simulink model "CORDIC"  (R2021a)
settings: Solver=VariableStepAuto  StartTime=0.0  StopTime=400  RelTol=1e-3
undefined symbols (not defined in the file or in its folder): AXI4, Lite
libraries: hdlBasic x776, xbsIndex_r4 x1
(part 1 of 7)
settings Model: Creator=jz118  LastModifiedBy=jz118

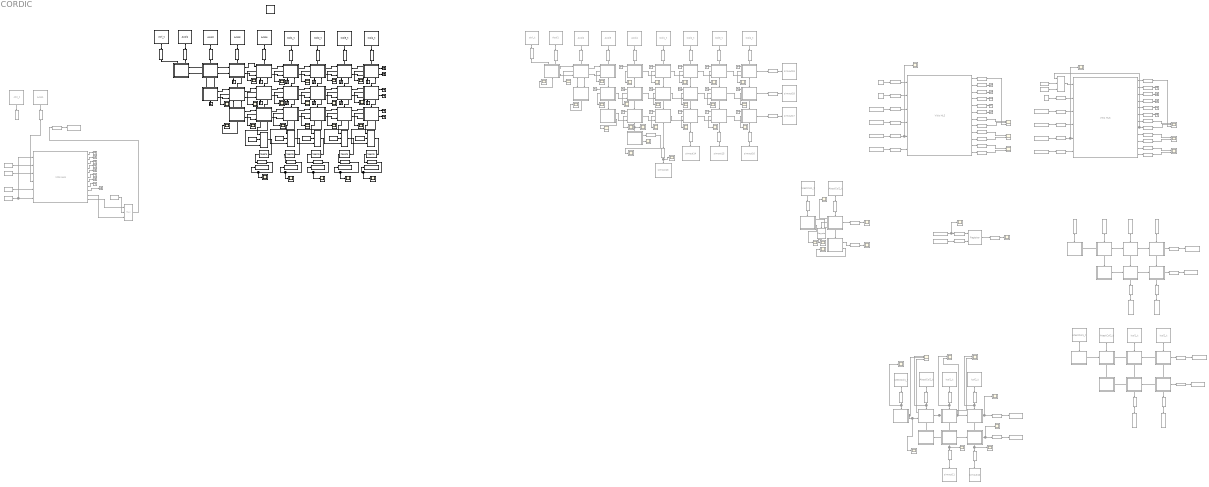
== system CORDIC ==
  " System Generator1" : xbsIndex_r4/ System Generator  Tag=genX  xilinxfamily=zynq  part=xc7z020  speed=-1  package=clg484  synthesis_tool=Vivado  clock_wrapper=Clock Enables  directory=./netlistA4  proj_type=Vivado  Synth_file=Vivado Synthesis Defaults  Impl_file=Vivado Implementation Defaults  testbench=off  simulink_period=1  sysclk_period=10  dcm_input_clock_period=10  incr_netlist=off  trim_vbits=Everywhere in SubSystem  dbl_ovrd=According to Block Masks  core_generation=According to Block Masks  run_coregen=off  deprecated_control=off  eval_field=0  block_type=sysgen
  Constant : hdlBasic/Constant  Commented=on  const=0  gui_display_data_type=Boolean  arith_type=Boolean  n_bits=16  bin_pt=14  preci_type=Single  exp_width=8  frac_width=24  explicit_period=off  period=1  XmcBlockStatus=1  maskContainerNames=tabcontainer1  block_type=constant  block_config=sysgen:Constant_config
  Constant1 : hdlBasic/Constant  Commented=on  const=1.0  gui_display_data_type=Boolean  arith_type=Boolean  n_bits=16  bin_pt=14  preci_type=Single  exp_width=8  frac_width=24  explicit_period=off  period=1  XmcBlockStatus=1  maskContainerNames=tabcontainer1  block_type=constant  block_config=sysgen:Constant_config
  Constant10 : hdlBasic/Constant  Commented=on  const=0  gui_display_data_type=Fixed-point  arith_type=Signed (2's comp)  n_bits=16  bin_pt=13  preci_type=Single  exp_width=8  frac_width=24  explicit_period=off  period=1  XmcBlockStatus=1  maskContainerNames=tabcontainer1  block_type=constant  block_config=sysgen:Constant_config
  Constant{4,6..8,11} (5 alike) : hdlBasic/Constant  const=0  gui_display_data_type=Fixed-point  arith_type=Signed (2's comp)  n_bits=16  bin_pt=13  preci_type=Single  exp_width=8  frac_width=24  explicit_period=off  period=1  XmcBlockStatus=1  maskContainerNames=tabcontainer1  block_type=constant  block_config=sysgen:Constant_config
  Constant12 : hdlBasic/Constant  Commented=on  const=0  gui_display_data_type=Boolean  arith_type=Boolean  n_bits=16  bin_pt=13  preci_type=Single  exp_width=8  frac_width=24  explicit_period=off  period=1  XmcBlockStatus=1  maskContainerNames=tabcontainer1  block_type=constant  block_config=sysgen:Constant_config
  Constant13 : hdlBasic/Constant  Commented=on  const=1  gui_display_data_type=Boolean  arith_type=Boolean  n_bits=16  bin_pt=13  preci_type=Single  exp_width=8  frac_width=24  explicit_period=off  period=1  XmcBlockStatus=1  maskContainerNames=tabcontainer1  block_type=constant  block_config=sysgen:Constant_config
  Constant14 : hdlBasic/Constant  Commented=on  const=0  gui_display_data_type=Fixed-point  arith_type=Signed (2's comp)  n_bits=16  bin_pt=13  preci_type=Single  exp_width=8  frac_width=24  explicit_period=off  period=1  XmcBlockStatus=1  maskContainerNames=tabcontainer1  block_type=constant  block_config=sysgen:Constant_config
  Constant2 : Constant  Commented=on
  Constant3 : Constant  Commented=on  Value=0
  Constant5 : Constant  Commented=on
  Constant9 : hdlBasic/Constant  Commented=on  const=0  gui_display_data_type=Fixed-point  arith_type=Signed (2's comp)  n_bits=16  bin_pt=13  preci_type=Single  exp_width=8  frac_width=24  explicit_period=off  period=1  XmcBlockStatus=1  maskContainerNames=tabcontainer1  block_type=constant  block_config=sysgen:Constant_config
  From Workspace1 : FromWorkspace  Commented=on  VariableName=y
  From Workspace10 : FromWorkspace  Commented=on  VariableName=AtestCol2_t
  From Workspace11 : FromWorkspace  Commented=on  VariableName=y
  From Workspace12 : FromWorkspace  Commented=on  VariableName=mode
  From Workspace13 : FromWorkspace  Commented=on  VariableName=theta
  From Workspace14 : FromWorkspace  Commented=on  VariableName=x
  From Workspace15 : FromWorkspace  Commented=on  VariableName=Icol1_t
  From Workspace16 : FromWorkspace  Commented=on  VariableName=Icol2_t
  From Workspace17 : FromWorkspace  Commented=on  VariableName=AtestCol1_t
  From Workspace18 : FromWorkspace  Commented=on  VariableName=AtestCol2_t
  From Workspace19 : FromWorkspace  Commented=on  VariableName=Icol1_t
  From Workspace2 : FromWorkspace  Commented=on  VariableName=mode
  From Workspace20 : FromWorkspace  Commented=on  VariableName=Icol2_t
  From Workspace21 : FromWorkspace  Commented=on  VariableName=regenable
  From Workspace22 : FromWorkspace  Commented=on  VariableName=regtest
  From Workspace23 : FromWorkspace  Commented=on  VariableName=AtestCol1_t
  From Workspace24 : FromWorkspace  Commented=on  VariableName=AtestCol2_t
  From Workspace25 : FromWorkspace  Commented=on  VariableName=Acol1
  From Workspace26 : FromWorkspace  Commented=on  VariableName=Acol2
  From Workspace27 : FromWorkspace  Commented=on  VariableName=Acol3
  From Workspace28 : FromWorkspace  Commented=on  VariableName=Acol4
  From Workspace29 : FromWorkspace  Commented=on  VariableName=Icol1_t
  From Workspace3 : FromWorkspace  Commented=on  VariableName=theta
  From Workspace30 : FromWorkspace  Commented=on  VariableName=Icol2_t
  From Workspace31 : FromWorkspace  Commented=on  VariableName=Icol3_t
  From Workspace32 : FromWorkspace  Commented=on  VariableName=Icol4_t
  From Workspace33 : FromWorkspace  Commented=on  VariableName=ctrl_t
  From Workspace34 : FromWorkspace  VariableName=Acol1
  From Workspace35 : FromWorkspace  VariableName=Acol2
  From Workspace36 : FromWorkspace  VariableName=Acol3
  From Workspace37 : FromWorkspace  VariableName=Acol4
  From Workspace38 : FromWorkspace  VariableName=ctrl_t
  From Workspace39 : FromWorkspace  VariableName=Icol1_t
  From Workspace4 : FromWorkspace  Commented=on  VariableName=x
  From Workspace40 : FromWorkspace  VariableName=Icol2_t
  From Workspace41 : FromWorkspace  VariableName=Icol3_t
  From Workspace42 : FromWorkspace  VariableName=Icol4_t
  From Workspace43 : FromWorkspace  Commented=on  VariableName=Acol1
  From Workspace44 : FromWorkspace  Commented=on  VariableName=ctrl_t
  From Workspace5 : FromWorkspace  Commented=on  VariableName=col1
  From Workspace6 : FromWorkspace  Commented=on  VariableName=col2
  From Workspace7 : FromWorkspace  Commented=on  VariableName=ident1
  From Workspace8 : FromWorkspace  Commented=on  VariableName=ident2
  From Workspace9 : FromWorkspace  Commented=on  VariableName=AtestCol1_t
  Gateway In{1,5,9..11} (5 alike) : hdlBasic/Gateway In  Commented=on  gui_display_data_type=Boolean  arith_type=Boolean  n_bits=16  bin_pt=3  preci_type=Single  exp_width=8  frac_width=24  rows=1  columns=1  quantization="Round  (unbiased: +/- Inf)"  overflow=Saturate  period=1  UseAsADC=off  ADCChannel='1'  interface=None  automatic_assignment=on  address_offset=hex2dec('00')  intf_name=''  intf_description=''  default_value=0  timing_constraint=None  locs_specified=off  LOCs={}  io_standard={}  inherit_from_input=off  hdl_port=on  XmcBlockStatus=1  maskContainerNames=group4  block_type=gatewayin  block_config=sysgen:gateway_in_config  block_width_w=590  block_height_w=620  block_width=640  block_height=850
  Gateway In{2..4,6..8,12..15,17..27} (21 alike) : hdlBasic/Gateway In  Commented=on  gui_display_data_type=Fixed-point  arith_type=Signed (2's comp)  n_bits=16  bin_pt=13  preci_type=Single  exp_width=8  frac_width=24  rows=1  columns=1  quantization="Round  (unbiased: +/- Inf)"  overflow=Saturate  period=1  UseAsADC=off  ADCChannel='1'  interface=None  automatic_assignment=on  address_offset=hex2dec('00')  intf_name=''  intf_description=''  default_value=0  timing_constraint=None  locs_specified=off  LOCs={}  io_standard={}  inherit_from_input=off  hdl_port=on  XmcBlockStatus=1  maskContainerNames=group4  block_type=gatewayin  block_config=sysgen:gateway_in_config  block_width_w=590  block_height_w=620  block_width=640  block_height=850
  Gateway In16 : hdlBasic/Gateway In  Commented=on  gui_display_data_type=Boolean  arith_type=Boolean  n_bits=16  bin_pt=13  preci_type=Single  exp_width=8  frac_width=24  rows=1  columns=1  quantization="Round  (unbiased: +/- Inf)"  overflow=Saturate  period=1  UseAsADC=off  ADCChannel='1'  interface=None  automatic_assignment=on  address_offset=hex2dec('00')  intf_name=''  intf_description=''  default_value=0  timing_constraint=None  locs_specified=off  LOCs={}  io_standard={}  inherit_from_input=off  hdl_port=on  XmcBlockStatus=1  maskContainerNames=group4  block_type=gatewayin  block_config=sysgen:gateway_in_config  block_width_w=590  block_height_w=620  block_width=640  block_height=850
  Gateway In28 : hdlBasic/Gateway In  Commented=on  gui_display_data_type=Boolean  arith_type=Boolean  n_bits=16  bin_pt=13  preci_type=Single  exp_width=8  frac_width=24  rows=1  columns=1  quantization="Round  (unbiased: +/- Inf)"  overflow=Saturate  period=1  UseAsADC=off  ADCChannel='1'  interface=None  automatic_assignment=on  address_offset=hex2dec('00')  intf_name=''  intf_description=''  default_value=0  timing_constraint=None  locs_specified=off  LOCs={}  io_standard={}  inherit_from_input=off  hdl_port=on  XmcBlockStatus=1  maskContainerNames=group4  block_type=gatewayin  block_config=sysgen:gateway_in_config  block_width_w=590  block_height_w=620  block_width=640  block_height=850
  Gateway In29 : hdlBasic/Gateway In  gui_display_data_type=Fixed-point  arith_type=Signed (2's comp)  n_bits=16  bin_pt=13  preci_type=Single  exp_width=8  frac_width=24  rows=1  columns=1  quantization="Round  (unbiased: +/- Inf)"  overflow=Saturate  period=1  UseAsADC=off  ADCChannel='1'  interface=AXI4-Lite  automatic_assignment=on  address_offset=hex2dec('00')  intf_name=''  intf_description='Acol1'  default_value=0  timing_constraint=None  locs_specified=off  LOCs={}  io_standard={}  inherit_from_input=off  hdl_port=on  XmcBlockStatus=1  maskContainerNames=group4  block_type=gatewayin  block_config=sysgen:gateway_in_config  block_width_w=590  block_height_w=620  block_width=640  block_height=850
  Gateway In30 : hdlBasic/Gateway In  gui_display_data_type=Fixed-point  arith_type=Signed (2's comp)  n_bits=16  bin_pt=13  preci_type=Single  exp_width=8  frac_width=24  rows=1  columns=1  quantization="Round  (unbiased: +/- Inf)"  overflow=Saturate  period=1  UseAsADC=off  ADCChannel='1'  interface=AXI4-Lite  automatic_assignment=on  address_offset=hex2dec('00')  intf_name=''  intf_description='Acol2'  default_value=0  timing_constraint=None  locs_specified=off  LOCs={}  io_standard={}  inherit_from_input=off  hdl_port=on  XmcBlockStatus=1  maskContainerNames=group4  block_type=gatewayin  block_config=sysgen:gateway_in_config  block_width_w=590  block_height_w=620  block_width=640  block_height=850
  Gateway In31 : hdlBasic/Gateway In  gui_display_data_type=Fixed-point  arith_type=Signed (2's comp)  n_bits=16  bin_pt=13  preci_type=Single  exp_width=8  frac_width=24  rows=1  columns=1  quantization="Round  (unbiased: +/- Inf)"  overflow=Saturate  period=1  UseAsADC=off  ADCChannel='1'  interface=AXI4-Lite  automatic_assignment=on  address_offset=hex2dec('00')  intf_name=''  intf_description='Acol3'  default_value=0  timing_constraint=None  locs_specified=off  LOCs={}  io_standard={}  inherit_from_input=off  hdl_port=on  XmcBlockStatus=1  maskContainerNames=group4  block_type=gatewayin  block_config=sysgen:gateway_in_config  block_width_w=590  block_height_w=620  block_width=640  block_height=850
  Gateway In32 : hdlBasic/Gateway In  gui_display_data_type=Fixed-point  arith_type=Signed (2's comp)  n_bits=16  bin_pt=13  preci_type=Single  exp_width=8  frac_width=24  rows=1  columns=1  quantization="Round  (unbiased: +/- Inf)"  overflow=Saturate  period=1  UseAsADC=off  ADCChannel='1'  interface=AXI4-Lite  automatic_assignment=on  address_offset=hex2dec('00')  intf_name=''  intf_description='Acol4'  default_value=0  timing_constraint=None  locs_specified=off  LOCs={}  io_standard={}  inherit_from_input=off  hdl_port=on  XmcBlockStatus=1  maskContainerNames=group4  block_type=gatewayin  block_config=sysgen:gateway_in_config  block_width_w=590  block_height_w=620  block_width=640  block_height=850
  Gateway In33 : hdlBasic/Gateway In  Commented=on  gui_display_data_type=Fixed-point  arith_type=Signed (2's comp)  n_bits=16  bin_pt=13  preci_type=Single  exp_width=8  frac_width=24  rows=1  columns=1  quantization="Round  (unbiased: +/- Inf)"  overflow=Saturate  period=1  UseAsADC=off  ADCChannel='1'  interface=AXI4-Lite  automatic_assignment=on  address_offset=hex2dec('00')  intf_name=''  intf_description='Acol1'  default_value=0  timing_constraint=None  locs_specified=off  LOCs={}  io_standard={}  inherit_from_input=off  hdl_port=on  XmcBlockStatus=1  maskContainerNames=group4  block_type=gatewayin  block_config=sysgen:gateway_in_config  block_width_w=590  block_height_w=620  block_width=640  block_height=850
  Gateway In34 : hdlBasic/Gateway In  gui_display_data_type=Fixed-point  arith_type=Signed (2's comp)  n_bits=16  bin_pt=13  preci_type=Single  exp_width=8  frac_width=24  rows=1  columns=1  quantization="Round  (unbiased: +/- Inf)"  overflow=Saturate  period=1  UseAsADC=off  ADCChannel='1'  interface=AXI4-Lite  automatic_assignment=on  address_offset=hex2dec('00')  intf_name=''  intf_description='Icol1_t'  default_value=0  timing_constraint=None  locs_specified=off  LOCs={}  io_standard={}  inherit_from_input=off  hdl_port=on  XmcBlockStatus=1  maskContainerNames=group4  block_type=gatewayin  block_config=sysgen:gateway_in_config  block_width_w=590  block_height_w=620  block_width=640  block_height=850
  Gateway In35 : hdlBasic/Gateway In  gui_display_data_type=Fixed-point  arith_type=Signed (2's comp)  n_bits=16  bin_pt=13  preci_type=Single  exp_width=8  frac_width=24  rows=1  columns=1  quantization="Round  (unbiased: +/- Inf)"  overflow=Saturate  period=1  UseAsADC=off  ADCChannel='1'  interface=AXI4-Lite  automatic_assignment=on  address_offset=hex2dec('00')  intf_name=''  intf_description='Icol2_t'  default_value=0  timing_constraint=None  locs_specified=off  LOCs={}  io_standard={}  inherit_from_input=off  hdl_port=on  XmcBlockStatus=1  maskContainerNames=group4  block_type=gatewayin  block_config=sysgen:gateway_in_config  block_width_w=590  block_height_w=620  block_width=640  block_height=850
  Gateway In36 : hdlBasic/Gateway In  gui_display_data_type=Fixed-point  arith_type=Signed (2's comp)  n_bits=16  bin_pt=13  preci_type=Single  exp_width=8  frac_width=24  rows=1  columns=1  quantization="Round  (unbiased: +/- Inf)"  overflow=Saturate  period=1  UseAsADC=off  ADCChannel='1'  interface=AXI4-Lite  automatic_assignment=on  address_offset=hex2dec('00')  intf_name=''  intf_description='Icol3_t'  default_value=0  timing_constraint=None  locs_specified=off  LOCs={}  io_standard={}  inherit_from_input=off  hdl_port=on  XmcBlockStatus=1  maskContainerNames=group4  block_type=gatewayin  block_config=sysgen:gateway_in_config  block_width_w=590  block_height_w=620  block_width=640  block_height=850
  Gateway In37 : hdlBasic/Gateway In  gui_display_data_type=Fixed-point  arith_type=Signed (2's comp)  n_bits=16  bin_pt=13  preci_type=Single  exp_width=8  frac_width=24  rows=1  columns=1  quantization="Round  (unbiased: +/- Inf)"  overflow=Saturate  period=1  UseAsADC=off  ADCChannel='1'  interface=AXI4-Lite  automatic_assignment=on  address_offset=hex2dec('00')  intf_name=''  intf_description='Icol4_t'  default_value=0  timing_constraint=None  locs_specified=off  LOCs={}  io_standard={}  inherit_from_input=off  hdl_port=on  XmcBlockStatus=1  maskContainerNames=group4  block_type=gatewayin  block_config=sysgen:gateway_in_config  block_width_w=590  block_height_w=620  block_width=640  block_height=850
  Gateway Out{,1..42,44..47} (47 alike) : hdlBasic/Gateway Out  Commented=on  inherit_from_input=off  hdl_port=on  rows=1  columns=1  UseAsDAC=off  DACChannel='1'  interface=None  automatic_assignment=on  address_offset=hex2dec('00')  intf_name=''  intf_description=''  timing_constraint=None  locs_specified=off  LOCs={}  io_standard={}  XmcBlockStatus=1  maskContainerNames=group4  block_type=gatewayout  block_config=sysgen:gateway_out_config  block_width_w=590  block_height_w=620  block_width=620  block_height=750
  Gateway Out43 : hdlBasic/Gateway Out  inherit_from_input=off  hdl_port=on  rows=1  columns=1  UseAsDAC=off  DACChannel='1'  interface=AXI4-Lite  automatic_assignment=on  address_offset=hex2dec('00')  intf_name=''  intf_description='R_4_4'  timing_constraint=None  locs_specified=off  LOCs={}  io_standard={}  XmcBlockStatus=1  maskContainerNames=group4  block_type=gatewayout  block_config=sysgen:gateway_out_config  block_width_w=590  block_height_w=620  block_width=620  block_height=750
  Gateway Out48 : hdlBasic/Gateway Out  inherit_from_input=off  hdl_port=on  rows=1  columns=1  UseAsDAC=off  DACChannel='1'  interface=AXI4-Lite  automatic_assignment=on  address_offset=hex2dec('00')  intf_name=''  intf_description='Q_4_1'  timing_constraint=None  locs_specified=off  LOCs={}  io_standard={}  XmcBlockStatus=1  maskContainerNames=group4  block_type=gatewayout  block_config=sysgen:gateway_out_config  block_width_w=590  block_height_w=620  block_width=620  block_height=750
  Gateway Out49 : hdlBasic/Gateway Out  inherit_from_input=off  hdl_port=on  rows=1  columns=1  UseAsDAC=off  DACChannel='1'  interface=AXI4-Lite  automatic_assignment=on  address_offset=hex2dec('00')  intf_name=''  intf_description='Q_4_2'  timing_constraint=None  locs_specified=off  LOCs={}  io_standard={}  XmcBlockStatus=1  maskContainerNames=group4  block_type=gatewayout  block_config=sysgen:gateway_out_config  block_width_w=590  block_height_w=620  block_width=620  block_height=750
  Gateway Out50 : hdlBasic/Gateway Out  inherit_from_input=off  hdl_port=on  rows=1  columns=1  UseAsDAC=off  DACChannel='1'  interface=AXI4-Lite  automatic_assignment=on  address_offset=hex2dec('00')  intf_name=''  intf_description='Q_4_3'  timing_constraint=None  locs_specified=off  LOCs={}  io_standard={}  XmcBlockStatus=1  maskContainerNames=group4  block_type=gatewayout  block_config=sysgen:gateway_out_config  block_width_w=590  block_height_w=620  block_width=620  block_height=750
  Gateway Out51 : hdlBasic/Gateway Out  inherit_from_input=off  hdl_port=on  rows=1  columns=1  UseAsDAC=off  DACChannel='1'  interface=AXI4-Lite  automatic_assignment=on  address_offset=hex2dec('00')  intf_name=''  intf_description='Q_4_4'  timing_constraint=None  locs_specified=off  LOCs={}  io_standard={}  XmcBlockStatus=1  maskContainerNames=group4  block_type=gatewayout  block_config=sysgen:gateway_out_config  block_width_w=590  block_height_w=620  block_width=620  block_height=750
  Gateway Out52 : hdlBasic/Gateway Out  Commented=on  inherit_from_input=off  hdl_port=on  rows=1  columns=1  UseAsDAC=off  DACChannel='1'  interface=AXI4-Lite  automatic_assignment=on  address_offset=hex2dec('00')  intf_name=''  intf_description='R_4_4'  timing_constraint=None  locs_specified=off  LOCs={}  io_standard={}  XmcBlockStatus=1  maskContainerNames=group4  block_type=gatewayout  block_config=sysgen:gateway_out_config  block_width_w=590  block_height_w=620  block_width=620  block_height=750
  Mux : hdlBasic/Mux  Commented=on  inputs=2  en=off  latency=1  precision=Full  arith_type=Unsigned  n_bits=16  bin_pt=14  quantization=Truncate  overflow=Wrap  XmcBlockStatus=1  maskContainerNames=tabcontainer1  block_type=mux  block_config=sysgen:Mux_config
  Mux{1..5} (5 alike) : hdlBasic/Mux  inputs=2  en=off  latency=1  precision=Full  arith_type=Unsigned  n_bits=16  bin_pt=14  quantization=Truncate  overflow=Wrap  XmcBlockStatus=1  maskContainerNames=tabcontainer1  block_type=mux  block_config=sysgen:Mux_config
  Mux6 : hdlBasic/Mux  Commented=on  inputs=2  en=off  latency=1  precision=Full  arith_type=Unsigned  n_bits=16  bin_pt=14  quantization=Truncate  overflow=Wrap  XmcBlockStatus=1  maskContainerNames=tabcontainer1  block_type=mux  block_config=sysgen:Mux_config
  Negate : hdlBasic/Negate  Commented=on  precision=Full  arith_type=Unsigned  n_bits=16  bin_pt=14  quantization=Truncate  overflow=Wrap  en=off  latency=0  XmcBlockStatus=1  maskContainerNames=tabcontainer1  block_type=negate  block_config=sysgen:Negate_config
  Negate{1..5} (5 alike) : hdlBasic/Negate  precision=Full  arith_type=Unsigned  n_bits=16  bin_pt=14  quantization=Truncate  overflow=Wrap  en=off  latency=0  XmcBlockStatus=1  maskContainerNames=tabcontainer1  block_type=negate  block_config=sysgen:Negate_config
  Register : hdlBasic/Register  Commented=on  init=0  rst=off  en=on  XmcBlockStatus=1  maskContainerNames=tabcontainer1  block_type=register  block_config=sysgen:Register_config
  Rotation : Subsystem  Commented=on
      settings: PortSchema="{\"entries\":[{\"content\":{\"sides\":[{\"content\":{\"connectorIds\":[\"In1\"]},\"type\":\"ConnectorPlacement.EquallySpacedRectSide\",\"uuid\":\"b989bfd3-647b-468d-a24b-67c5817c2fb9\"},{\"content\":{\"connectorIds\":[\"Out1\"],\"side\":\"RIGHT\"},\"type\":\"ConnectorPlacement.EquallySpacedRectSide\",\"uuid\":\"15839450-c6b9-4b4c-b490-793a0225ad70\"},{\"content\":{\"connectorIds\":[\"In2\"],\"side\":\"TOP\"},\"type\":\"ConnectorPlacement.EquallySpacedRectSide\",\"uuid\":\"69a0ff69-1754-49ce-bc12-3d58954b90b5\"},{\"content\":{\"connectorIds\":[\"Out2\"],\"side\":\"BOTTOM\"},\"type\":\"ConnectorPlacement.EquallySpacedRectSide\",\"uuid\":\"c7c95c77-bae3-47b7-a54f-9afc9f4e7b60\"}]},\"type\":\"ConnectorPlacement.EquallySpacedConnector\",\"uuid\":\"47487c21-2009-4dc3-9515-f1b42d882620\"}],\"packageUris\":[\"http://schema.mathworks.com/mf0/Connector/R2020b\"],\"version\":\"1.0\"}"
  Rotation1 : Subsystem  Commented=on
      settings: PortSchema="{\"entries\":[{\"content\":{\"sides\":[{\"content\":{\"connectorIds\":[\"In1\"]},\"type\":\"ConnectorPlacement.EquallySpacedRectSide\",\"uuid\":\"b989bfd3-647b-468d-a24b-67c5817c2fb9\"},{\"content\":{\"connectorIds\":[\"Out1\"],\"side\":\"RIGHT\"},\"type\":\"ConnectorPlacement.EquallySpacedRectSide\",\"uuid\":\"15839450-c6b9-4b4c-b490-793a0225ad70\"},{\"content\":{\"connectorIds\":[\"In2\"],\"side\":\"TOP\"},\"type\":\"ConnectorPlacement.EquallySpacedRectSide\",\"uuid\":\"69a0ff69-1754-49ce-bc12-3d58954b90b5\"},{\"content\":{\"connectorIds\":[\"Out2\"],\"side\":\"BOTTOM\"},\"type\":\"ConnectorPlacement.EquallySpacedRectSide\",\"uuid\":\"c7c95c77-bae3-47b7-a54f-9afc9f4e7b60\"}]},\"type\":\"ConnectorPlacement.EquallySpacedConnector\",\"uuid\":\"47487c21-2009-4dc3-9515-f1b42d882620\"}],\"packageUris\":[\"http://schema.mathworks.com/mf0/Connector/R2020b\"],\"version\":\"1.0\"}"
  Rotation10 : Subsystem  Commented=on
      settings: PortSchema="{\"entries\":[{\"content\":{\"sides\":[{\"content\":{\"connectorIds\":[\"Out3\",\"In1\"]},\"type\":\"ConnectorPlacement.EquallySpacedRectSide\",\"uuid\":\"b989bfd3-647b-468d-a24b-67c5817c2fb9\"},{\"content\":{\"connectorIds\":[\"Out1\"],\"side\":\"RIGHT\"},\"type\":\"ConnectorPlacement.EquallySpacedRectSide\",\"uuid\":\"15839450-c6b9-4b4c-b490-793a0225ad70\"},{\"content\":{\"connectorIds\":[\"In2\"],\"side\":\"TOP\"},\"type\":\"ConnectorPlacement.EquallySpacedRectSide\",\"uuid\":\"69a0ff69-1754-49ce-bc12-3d58954b90b5\"},{\"content\":{\"connectorIds\":[\"Out2\"],\"side\":\"BOTTOM\"},\"type\":\"ConnectorPlacement.EquallySpacedRectSide\",\"uuid\":\"c7c95c77-bae3-47b7-a54f-9afc9f4e7b60\"}]},\"type\":\"ConnectorPlacement.EquallySpacedConnector\",\"uuid\":\"47487c21-2009-4dc3-9515-f1b42d882620\"}],\"packageUris\":[\"http://schema.mathworks.com/mf0/Connector/R2020b\"],\"version\":\"1.0\"}"
  Rotation11 : Subsystem  Commented=on
      settings: PortSchema="{\"entries\":[{\"content\":{\"sides\":[{\"content\":{\"connectorIds\":[\"In1\"]},\"type\":\"ConnectorPlacement.EquallySpacedRectSide\",\"uuid\":\"b989bfd3-647b-468d-a24b-67c5817c2fb9\"},{\"content\":{\"connectorIds\":[\"Out1\"],\"side\":\"RIGHT\"},\"type\":\"ConnectorPlacement.EquallySpacedRectSide\",\"uuid\":\"15839450-c6b9-4b4c-b490-793a0225ad70\"},{\"content\":{\"connectorIds\":[\"In2\"],\"side\":\"TOP\"},\"type\":\"ConnectorPlacement.EquallySpacedRectSide\",\"uuid\":\"69a0ff69-1754-49ce-bc12-3d58954b90b5\"},{\"content\":{\"connectorIds\":[\"Out2\"],\"side\":\"BOTTOM\"},\"type\":\"ConnectorPlacement.EquallySpacedRectSide\",\"uuid\":\"c7c95c77-bae3-47b7-a54f-9afc9f4e7b60\"}]},\"type\":\"ConnectorPlacement.EquallySpacedConnector\",\"uuid\":\"47487c21-2009-4dc3-9515-f1b42d882620\"}],\"packageUris\":[\"http://schema.mathworks.com/mf0/Connector/R2020b\"],\"version\":\"1.0\"}"
  Rotation12 : Subsystem  Commented=on
      settings: PortSchema="{\"entries\":[{\"content\":{\"sides\":[{\"content\":{\"connectorIds\":[\"In1\"]},\"type\":\"ConnectorPlacement.EquallySpacedRectSide\",\"uuid\":\"b989bfd3-647b-468d-a24b-67c5817c2fb9\"},{\"content\":{\"connectorIds\":[\"Out1\"],\"side\":\"RIGHT\"},\"type\":\"ConnectorPlacement.EquallySpacedRectSide\",\"uuid\":\"15839450-c6b9-4b4c-b490-793a0225ad70\"},{\"content\":{\"connectorIds\":[\"In2\"],\"side\":\"TOP\"},\"type\":\"ConnectorPlacement.EquallySpacedRectSide\",\"uuid\":\"69a0ff69-1754-49ce-bc12-3d58954b90b5\"},{\"content\":{\"connectorIds\":[\"Out2\"],\"side\":\"BOTTOM\"},\"type\":\"ConnectorPlacement.EquallySpacedRectSide\",\"uuid\":\"c7c95c77-bae3-47b7-a54f-9afc9f4e7b60\"}]},\"type\":\"ConnectorPlacement.EquallySpacedConnector\",\"uuid\":\"47487c21-2009-4dc3-9515-f1b42d882620\"}],\"packageUris\":[\"http://schema.mathworks.com/mf0/Connector/R2020b\"],\"version\":\"1.0\"}"
  Rotation13 : Subsystem  Commented=on
      settings: PortSchema="{\"entries\":[{\"content\":{\"sides\":[{\"content\":{\"connectorIds\":[\"Out3\",\"Out4\",\"In1\"]},\"type\":\"ConnectorPlacement.EquallySpacedRectSide\",\"uuid\":\"b989bfd3-647b-468d-a24b-67c5817c2fb9\"},{\"content\":{\"connectorIds\":[\"Out1\"],\"side\":\"RIGHT\"},\"type\":\"ConnectorPlacement.EquallySpacedRectSide\",\"uuid\":\"15839450-c6b9-4b4c-b490-793a0225ad70\"},{\"content\":{\"connectorIds\":[\"In2\"],\"side\":\"TOP\"},\"type\":\"ConnectorPlacement.EquallySpacedRectSide\",\"uuid\":\"69a0ff69-1754-49ce-bc12-3d58954b90b5\"},{\"content\":{\"connectorIds\":[\"Out2\"],\"side\":\"BOTTOM\"},\"type\":\"ConnectorPlacement.EquallySpacedRectSide\",\"uuid\":\"c7c95c77-bae3-47b7-a54f-9afc9f4e7b60\"}]},\"type\":\"ConnectorPlacement.EquallySpacedConnector\",\"uuid\":\"47487c21-2009-4dc3-9515-f1b42d882620\"}],\"packageUris\":[\"http://schema.mathworks.com/mf0/Connector/R2020b\"],\"version\":\"1.0\"}"
  Rotation14 : Subsystem  Commented=on
      settings: PortSchema="{\"entries\":[{\"content\":{\"sides\":[{\"content\":{\"connectorIds\":[\"In1\"]},\"type\":\"ConnectorPlacement.EquallySpacedRectSide\",\"uuid\":\"b989bfd3-647b-468d-a24b-67c5817c2fb9\"},{\"content\":{\"connectorIds\":[\"Out1\"],\"side\":\"RIGHT\"},\"type\":\"ConnectorPlacement.EquallySpacedRectSide\",\"uuid\":\"15839450-c6b9-4b4c-b490-793a0225ad70\"},{\"content\":{\"connectorIds\":[\"In2\"],\"side\":\"TOP\"},\"type\":\"ConnectorPlacement.EquallySpacedRectSide\",\"uuid\":\"69a0ff69-1754-49ce-bc12-3d58954b90b5\"},{\"content\":{\"connectorIds\":[\"Out2\"],\"side\":\"BOTTOM\"},\"type\":\"ConnectorPlacement.EquallySpacedRectSide\",\"uuid\":\"c7c95c77-bae3-47b7-a54f-9afc9f4e7b60\"}]},\"type\":\"ConnectorPlacement.EquallySpacedConnector\",\"uuid\":\"47487c21-2009-4dc3-9515-f1b42d882620\"}],\"packageUris\":[\"http://schema.mathworks.com/mf0/Connector/R2020b\"],\"version\":\"1.0\"}"
  Rotation15 : Subsystem  Commented=on
      settings: PortSchema="{\"entries\":[{\"content\":{\"sides\":[{\"content\":{\"connectorIds\":[\"In1\"]},\"type\":\"ConnectorPlacement.EquallySpacedRectSide\",\"uuid\":\"b989bfd3-647b-468d-a24b-67c5817c2fb9\"},{\"content\":{\"connectorIds\":[\"Out1\"],\"side\":\"RIGHT\"},\"type\":\"ConnectorPlacement.EquallySpacedRectSide\",\"uuid\":\"15839450-c6b9-4b4c-b490-793a0225ad70\"},{\"content\":{\"connectorIds\":[\"In2\"],\"side\":\"TOP\"},\"type\":\"ConnectorPlacement.EquallySpacedRectSide\",\"uuid\":\"69a0ff69-1754-49ce-bc12-3d58954b90b5\"},{\"content\":{\"connectorIds\":[\"Out2\"],\"side\":\"BOTTOM\"},\"type\":\"ConnectorPlacement.EquallySpacedRectSide\",\"uuid\":\"c7c95c77-bae3-47b7-a54f-9afc9f4e7b60\"}]},\"type\":\"ConnectorPlacement.EquallySpacedConnector\",\"uuid\":\"47487c21-2009-4dc3-9515-f1b42d882620\"}],\"packageUris\":[\"http://schema.mathworks.com/mf0/Connector/R2020b\"],\"version\":\"1.0\"}"
  Rotation16 : Subsystem  Commented=on
      settings: PortSchema="{\"entries\":[{\"content\":{\"sides\":[{\"content\":{\"connectorIds\":[\"In1\",\"Out5\",\"In2\"]},\"type\":\"ConnectorPlacement.EquallySpacedRectSide\",\"uuid\":\"b989bfd3-647b-468d-a24b-67c5817c2fb9\"},{\"content\":{\"connectorIds\":[\"Out1\",\"Out2\"],\"side\":\"RIGHT\"},\"type\":\"ConnectorPlacement.EquallySpacedRectSide\",\"uuid\":\"15839450-c6b9-4b4c-b490-793a0225ad70\"},{\"content\":{\"connectorIds\":[\"In3\"],\"side\":\"TOP\"},\"type\":\"ConnectorPlacement.EquallySpacedRectSide\",\"uuid\":\"69a0ff69-1754-49ce-bc12-3d58954b90b5\"},{\"content\":{\"connectorIds\":[\"Out3\",\"Out4\"],\"side\":\"BOTTOM\"},\"type\":\"ConnectorPlacement.EquallySpacedRectSide\",\"uuid\":\"c7c95c77-bae3-47b7-a54f-9afc9f4e7b60\"}]},\"type\":\"ConnectorPlacement.EquallySpacedConnector\",\"uuid\":\"47487c21-2009-4dc3-9515-f1b42d882620\"}],\"packageUris\":[\"http://schema.mathworks.com/mf0/Connector/R2020b\"],\"version\":\"1.0\"}"
  Rotation17 : Subsystem  Commented=on
      settings: PortSchema="{\"entries\":[{\"content\":{\"sides\":[{\"content\":{\"connectorIds\":[\"In1\",\"Out4\",\"In2\"]},\"type\":\"ConnectorPlacement.EquallySpacedRectSide\",\"uuid\":\"b989bfd3-647b-468d-a24b-67c5817c2fb9\"},{\"content\":{\"connectorIds\":[\"Out1\",\"Out2\"],\"side\":\"RIGHT\"},\"type\":\"ConnectorPlacement.EquallySpacedRectSide\",\"uuid\":\"15839450-c6b9-4b4c-b490-793a0225ad70\"},{\"content\":{\"connectorIds\":[\"In3\"],\"side\":\"TOP\"},\"type\":\"ConnectorPlacement.EquallySpacedRectSide\",\"uuid\":\"69a0ff69-1754-49ce-bc12-3d58954b90b5\"},{\"content\":{\"connectorIds\":[\"Out3\"],\"side\":\"BOTTOM\"},\"type\":\"ConnectorPlacement.EquallySpacedRectSide\",\"uuid\":\"c7c95c77-bae3-47b7-a54f-9afc9f4e7b60\"}]},\"type\":\"ConnectorPlacement.EquallySpacedConnector\",\"uuid\":\"47487c21-2009-4dc3-9515-f1b42d882620\"}],\"packageUris\":[\"http://schema.mathworks.com/mf0/Connector/R2020b\"],\"version\":\"1.0\"}"
  Rotation18 : Subsystem  Commented=on
      settings: PortSchema="{\"entries\":[{\"content\":{\"sides\":[{\"content\":{\"connectorIds\":[\"Out3\",\"Out4\",\"In1\"]},\"type\":\"ConnectorPlacement.EquallySpacedRectSide\",\"uuid\":\"b989bfd3-647b-468d-a24b-67c5817c2fb9\"},{\"content\":{\"connectorIds\":[\"Out1\"],\"side\":\"RIGHT\"},\"type\":\"ConnectorPlacement.EquallySpacedRectSide\",\"uuid\":\"15839450-c6b9-4b4c-b490-793a0225ad70\"},{\"content\":{\"connectorIds\":[\"In2\"],\"side\":\"TOP\"},\"type\":\"ConnectorPlacement.EquallySpacedRectSide\",\"uuid\":\"69a0ff69-1754-49ce-bc12-3d58954b90b5\"},{\"content\":{\"connectorIds\":[\"Out2\"],\"side\":\"BOTTOM\"},\"type\":\"ConnectorPlacement.EquallySpacedRectSide\",\"uuid\":\"c7c95c77-bae3-47b7-a54f-9afc9f4e7b60\"}]},\"type\":\"ConnectorPlacement.EquallySpacedConnector\",\"uuid\":\"47487c21-2009-4dc3-9515-f1b42d882620\"}],\"packageUris\":[\"http://schema.mathworks.com/mf0/Connector/R2020b\"],\"version\":\"1.0\"}"
  Rotation19 : Subsystem  Commented=on
      settings: PortSchema="{\"entries\":[{\"content\":{\"sides\":[{\"content\":{\"connectorIds\":[\"Out3\",\"Out4\",\"In1\"]},\"type\":\"ConnectorPlacement.EquallySpacedRectSide\",\"uuid\":\"b989bfd3-647b-468d-a24b-67c5817c2fb9\"},{\"content\":{\"connectorIds\":[\"Out1\"],\"side\":\"RIGHT\"},\"type\":\"ConnectorPlacement.EquallySpacedRectSide\",\"uuid\":\"15839450-c6b9-4b4c-b490-793a0225ad70\"},{\"content\":{\"connectorIds\":[\"In2\"],\"side\":\"TOP\"},\"type\":\"ConnectorPlacement.EquallySpacedRectSide\",\"uuid\":\"69a0ff69-1754-49ce-bc12-3d58954b90b5\"},{\"content\":{\"connectorIds\":[\"Out2\"],\"side\":\"BOTTOM\"},\"type\":\"ConnectorPlacement.EquallySpacedRectSide\",\"uuid\":\"c7c95c77-bae3-47b7-a54f-9afc9f4e7b60\"}]},\"type\":\"ConnectorPlacement.EquallySpacedConnector\",\"uuid\":\"47487c21-2009-4dc3-9515-f1b42d882620\"}],\"packageUris\":[\"http://schema.mathworks.com/mf0/Connector/R2020b\"],\"version\":\"1.0\"}"
  Rotation2 : Subsystem  Commented=on
      settings: PortSchema="{\"entries\":[{\"content\":{\"sides\":[{\"content\":{\"connectorIds\":[\"In1\"]},\"type\":\"ConnectorPlacement.EquallySpacedRectSide\",\"uuid\":\"b989bfd3-647b-468d-a24b-67c5817c2fb9\"},{\"content\":{\"connectorIds\":[\"Out1\"],\"side\":\"RIGHT\"},\"type\":\"ConnectorPlacement.EquallySpacedRectSide\",\"uuid\":\"15839450-c6b9-4b4c-b490-793a0225ad70\"},{\"content\":{\"connectorIds\":[\"In2\"],\"side\":\"TOP\"},\"type\":\"ConnectorPlacement.EquallySpacedRectSide\",\"uuid\":\"69a0ff69-1754-49ce-bc12-3d58954b90b5\"},{\"content\":{\"connectorIds\":[\"Out2\"],\"side\":\"BOTTOM\"},\"type\":\"ConnectorPlacement.EquallySpacedRectSide\",\"uuid\":\"c7c95c77-bae3-47b7-a54f-9afc9f4e7b60\"}]},\"type\":\"ConnectorPlacement.EquallySpacedConnector\",\"uuid\":\"47487c21-2009-4dc3-9515-f1b42d882620\"}],\"packageUris\":[\"http://schema.mathworks.com/mf0/Connector/R2020b\"],\"version\":\"1.0\"}"
  Rotation20 : Subsystem  Commented=on
      settings: PortSchema="{\"entries\":[{\"content\":{\"sides\":[{\"content\":{\"connectorIds\":[\"Out3\",\"Out4\",\"In1\"]},\"type\":\"ConnectorPlacement.EquallySpacedRectSide\",\"uuid\":\"b989bfd3-647b-468d-a24b-67c5817c2fb9\"},{\"content\":{\"connectorIds\":[\"Out1\"],\"side\":\"RIGHT\"},\"type\":\"ConnectorPlacement.EquallySpacedRectSide\",\"uuid\":\"15839450-c6b9-4b4c-b490-793a0225ad70\"},{\"content\":{\"connectorIds\":[\"In2\"],\"side\":\"TOP\"},\"type\":\"ConnectorPlacement.EquallySpacedRectSide\",\"uuid\":\"69a0ff69-1754-49ce-bc12-3d58954b90b5\"},{\"content\":{\"connectorIds\":[\"Out2\"],\"side\":\"BOTTOM\"},\"type\":\"ConnectorPlacement.EquallySpacedRectSide\",\"uuid\":\"c7c95c77-bae3-47b7-a54f-9afc9f4e7b60\"}]},\"type\":\"ConnectorPlacement.EquallySpacedConnector\",\"uuid\":\"47487c21-2009-4dc3-9515-f1b42d882620\"}],\"packageUris\":[\"http://schema.mathworks.com/mf0/Connector/R2020b\"],\"version\":\"1.0\"}"
  Rotation21 : Subsystem  Commented=on
      settings: PortSchema="{\"entries\":[{\"content\":{\"sides\":[{\"content\":{\"connectorIds\":[\"Out3\",\"Out4\",\"In1\"]},\"type\":\"ConnectorPlacement.EquallySpacedRectSide\",\"uuid\":\"b989bfd3-647b-468d-a24b-67c5817c2fb9\"},{\"content\":{\"connectorIds\":[\"Out1\"],\"side\":\"RIGHT\"},\"type\":\"ConnectorPlacement.EquallySpacedRectSide\",\"uuid\":\"15839450-c6b9-4b4c-b490-793a0225ad70\"},{\"content\":{\"connectorIds\":[\"In2\"],\"side\":\"TOP\"},\"type\":\"ConnectorPlacement.EquallySpacedRectSide\",\"uuid\":\"69a0ff69-1754-49ce-bc12-3d58954b90b5\"},{\"content\":{\"connectorIds\":[\"Out2\"],\"side\":\"BOTTOM\"},\"type\":\"ConnectorPlacement.EquallySpacedRectSide\",\"uuid\":\"c7c95c77-bae3-47b7-a54f-9afc9f4e7b60\"}]},\"type\":\"ConnectorPlacement.EquallySpacedConnector\",\"uuid\":\"47487c21-2009-4dc3-9515-f1b42d882620\"}],\"packageUris\":[\"http://schema.mathworks.com/mf0/Connector/R2020b\"],\"version\":\"1.0\"}"
  Rotation22 : Subsystem  Commented=on
      settings: PortSchema="{\"entries\":[{\"content\":{\"sides\":[{\"content\":{\"connectorIds\":[\"Out3\",\"Out4\",\"In1\"]},\"type\":\"ConnectorPlacement.EquallySpacedRectSide\",\"uuid\":\"b989bfd3-647b-468d-a24b-67c5817c2fb9\"},{\"content\":{\"connectorIds\":[\"Out1\"],\"side\":\"RIGHT\"},\"type\":\"ConnectorPlacement.EquallySpacedRectSide\",\"uuid\":\"15839450-c6b9-4b4c-b490-793a0225ad70\"},{\"content\":{\"connectorIds\":[\"In2\"],\"side\":\"TOP\"},\"type\":\"ConnectorPlacement.EquallySpacedRectSide\",\"uuid\":\"69a0ff69-1754-49ce-bc12-3d58954b90b5\"},{\"content\":{\"connectorIds\":[\"Out2\"],\"side\":\"BOTTOM\"},\"type\":\"ConnectorPlacement.EquallySpacedRectSide\",\"uuid\":\"c7c95c77-bae3-47b7-a54f-9afc9f4e7b60\"}]},\"type\":\"ConnectorPlacement.EquallySpacedConnector\",\"uuid\":\"47487c21-2009-4dc3-9515-f1b42d882620\"}],\"packageUris\":[\"http://schema.mathworks.com/mf0/Connector/R2020b\"],\"version\":\"1.0\"}"
  Rotation23 : Subsystem  Commented=on
      settings: PortSchema="{\"entries\":[{\"content\":{\"sides\":[{\"content\":{\"connectorIds\":[\"Out3\",\"Out4\",\"In1\"]},\"type\":\"ConnectorPlacement.EquallySpacedRectSide\",\"uuid\":\"b989bfd3-647b-468d-a24b-67c5817c2fb9\"},{\"content\":{\"connectorIds\":[\"Out1\"],\"side\":\"RIGHT\"},\"type\":\"ConnectorPlacement.EquallySpacedRectSide\",\"uuid\":\"15839450-c6b9-4b4c-b490-793a0225ad70\"},{\"content\":{\"connectorIds\":[\"In2\"],\"side\":\"TOP\"},\"type\":\"ConnectorPlacement.EquallySpacedRectSide\",\"uuid\":\"69a0ff69-1754-49ce-bc12-3d58954b90b5\"},{\"content\":{\"connectorIds\":[\"Out2\"],\"side\":\"BOTTOM\"},\"type\":\"ConnectorPlacement.EquallySpacedRectSide\",\"uuid\":\"c7c95c77-bae3-47b7-a54f-9afc9f4e7b60\"}]},\"type\":\"ConnectorPlacement.EquallySpacedConnector\",\"uuid\":\"47487c21-2009-4dc3-9515-f1b42d882620\"}],\"packageUris\":[\"http://schema.mathworks.com/mf0/Connector/R2020b\"],\"version\":\"1.0\"}"
  Rotation24 : Subsystem  Commented=on
      settings: PortSchema="{\"entries\":[{\"content\":{\"sides\":[{\"content\":{\"connectorIds\":[\"Out3\",\"Out4\",\"In1\"]},\"type\":\"ConnectorPlacement.EquallySpacedRectSide\",\"uuid\":\"b989bfd3-647b-468d-a24b-67c5817c2fb9\"},{\"content\":{\"connectorIds\":[\"Out1\"],\"side\":\"RIGHT\"},\"type\":\"ConnectorPlacement.EquallySpacedRectSide\",\"uuid\":\"15839450-c6b9-4b4c-b490-793a0225ad70\"},{\"content\":{\"connectorIds\":[\"In2\"],\"side\":\"TOP\"},\"type\":\"ConnectorPlacement.EquallySpacedRectSide\",\"uuid\":\"69a0ff69-1754-49ce-bc12-3d58954b90b5\"},{\"content\":{\"connectorIds\":[\"Out2\"],\"side\":\"BOTTOM\"},\"type\":\"ConnectorPlacement.EquallySpacedRectSide\",\"uuid\":\"c7c95c77-bae3-47b7-a54f-9afc9f4e7b60\"}]},\"type\":\"ConnectorPlacement.EquallySpacedConnector\",\"uuid\":\"47487c21-2009-4dc3-9515-f1b42d882620\"}],\"packageUris\":[\"http://schema.mathworks.com/mf0/Connector/R2020b\"],\"version\":\"1.0\"}"
  Rotation25 : Subsystem  Commented=on
      settings: PortSchema="{\"entries\":[{\"content\":{\"sides\":[{\"content\":{\"connectorIds\":[\"Out3\",\"Out4\",\"In1\"]},\"type\":\"ConnectorPlacement.EquallySpacedRectSide\",\"uuid\":\"b989bfd3-647b-468d-a24b-67c5817c2fb9\"},{\"content\":{\"connectorIds\":[\"Out1\"],\"side\":\"RIGHT\"},\"type\":\"ConnectorPlacement.EquallySpacedRectSide\",\"uuid\":\"15839450-c6b9-4b4c-b490-793a0225ad70\"},{\"content\":{\"connectorIds\":[\"In2\"],\"side\":\"TOP\"},\"type\":\"ConnectorPlacement.EquallySpacedRectSide\",\"uuid\":\"69a0ff69-1754-49ce-bc12-3d58954b90b5\"},{\"content\":{\"connectorIds\":[\"Out2\"],\"side\":\"BOTTOM\"},\"type\":\"ConnectorPlacement.EquallySpacedRectSide\",\"uuid\":\"c7c95c77-bae3-47b7-a54f-9afc9f4e7b60\"}]},\"type\":\"ConnectorPlacement.EquallySpacedConnector\",\"uuid\":\"47487c21-2009-4dc3-9515-f1b42d882620\"}],\"packageUris\":[\"http://schema.mathworks.com/mf0/Connector/R2020b\"],\"version\":\"1.0\"}"
  Rotation26 : Subsystem  Commented=on
      settings: PortSchema="{\"entries\":[{\"content\":{\"sides\":[{\"content\":{\"connectorIds\":[\"Out3\",\"Out4\",\"In1\"]},\"type\":\"ConnectorPlacement.EquallySpacedRectSide\",\"uuid\":\"b989bfd3-647b-468d-a24b-67c5817c2fb9\"},{\"content\":{\"connectorIds\":[\"Out1\"],\"side\":\"RIGHT\"},\"type\":\"ConnectorPlacement.EquallySpacedRectSide\",\"uuid\":\"15839450-c6b9-4b4c-b490-793a0225ad70\"},{\"content\":{\"connectorIds\":[\"In2\"],\"side\":\"TOP\"},\"type\":\"ConnectorPlacement.EquallySpacedRectSide\",\"uuid\":\"69a0ff69-1754-49ce-bc12-3d58954b90b5\"},{\"content\":{\"connectorIds\":[\"Out2\"],\"side\":\"BOTTOM\"},\"type\":\"ConnectorPlacement.EquallySpacedRectSide\",\"uuid\":\"c7c95c77-bae3-47b7-a54f-9afc9f4e7b60\"}]},\"type\":\"ConnectorPlacement.EquallySpacedConnector\",\"uuid\":\"47487c21-2009-4dc3-9515-f1b42d882620\"}],\"packageUris\":[\"http://schema.mathworks.com/mf0/Connector/R2020b\"],\"version\":\"1.0\"}"
  Rotation27 : Subsystem  Commented=on
      settings: PortSchema="{\"entries\":[{\"content\":{\"sides\":[{\"content\":{\"connectorIds\":[\"Out3\",\"Out4\",\"In1\"]},\"type\":\"ConnectorPlacement.EquallySpacedRectSide\",\"uuid\":\"b989bfd3-647b-468d-a24b-67c5817c2fb9\"},{\"content\":{\"connectorIds\":[\"Out1\"],\"side\":\"RIGHT\"},\"type\":\"ConnectorPlacement.EquallySpacedRectSide\",\"uuid\":\"15839450-c6b9-4b4c-b490-793a0225ad70\"},{\"content\":{\"connectorIds\":[\"In2\"],\"side\":\"TOP\"},\"type\":\"ConnectorPlacement.EquallySpacedRectSide\",\"uuid\":\"69a0ff69-1754-49ce-bc12-3d58954b90b5\"},{\"content\":{\"connectorIds\":[\"Out2\"],\"side\":\"BOTTOM\"},\"type\":\"ConnectorPlacement.EquallySpacedRectSide\",\"uuid\":\"c7c95c77-bae3-47b7-a54f-9afc9f4e7b60\"}]},\"type\":\"ConnectorPlacement.EquallySpacedConnector\",\"uuid\":\"47487c21-2009-4dc3-9515-f1b42d882620\"}],\"packageUris\":[\"http://schema.mathworks.com/mf0/Connector/R2020b\"],\"version\":\"1.0\"}"
  Rotation28 : Subsystem  Commented=on
      settings: PortSchema="{\"entries\":[{\"content\":{\"sides\":[{\"content\":{\"connectorIds\":[\"Out3\",\"Out4\",\"In1\"]},\"type\":\"ConnectorPlacement.EquallySpacedRectSide\",\"uuid\":\"b989bfd3-647b-468d-a24b-67c5817c2fb9\"},{\"content\":{\"connectorIds\":[\"Out1\"],\"side\":\"RIGHT\"},\"type\":\"ConnectorPlacement.EquallySpacedRectSide\",\"uuid\":\"15839450-c6b9-4b4c-b490-793a0225ad70\"},{\"content\":{\"connectorIds\":[\"In2\"],\"side\":\"TOP\"},\"type\":\"ConnectorPlacement.EquallySpacedRectSide\",\"uuid\":\"69a0ff69-1754-49ce-bc12-3d58954b90b5\"},{\"content\":{\"connectorIds\":[\"Out2\"],\"side\":\"BOTTOM\"},\"type\":\"ConnectorPlacement.EquallySpacedRectSide\",\"uuid\":\"c7c95c77-bae3-47b7-a54f-9afc9f4e7b60\"}]},\"type\":\"ConnectorPlacement.EquallySpacedConnector\",\"uuid\":\"47487c21-2009-4dc3-9515-f1b42d882620\"}],\"packageUris\":[\"http://schema.mathworks.com/mf0/Connector/R2020b\"],\"version\":\"1.0\"}"
  Rotation29 : Subsystem  Commented=on
      settings: PortSchema="{\"entries\":[{\"content\":{\"sides\":[{\"content\":{\"connectorIds\":[\"Out3\",\"Out4\",\"In1\"]},\"type\":\"ConnectorPlacement.EquallySpacedRectSide\",\"uuid\":\"b989bfd3-647b-468d-a24b-67c5817c2fb9\"},{\"content\":{\"connectorIds\":[\"Out1\"],\"side\":\"RIGHT\"},\"type\":\"ConnectorPlacement.EquallySpacedRectSide\",\"uuid\":\"15839450-c6b9-4b4c-b490-793a0225ad70\"},{\"content\":{\"connectorIds\":[\"In2\"],\"side\":\"TOP\"},\"type\":\"ConnectorPlacement.EquallySpacedRectSide\",\"uuid\":\"69a0ff69-1754-49ce-bc12-3d58954b90b5\"},{\"content\":{\"connectorIds\":[\"Out2\"],\"side\":\"BOTTOM\"},\"type\":\"ConnectorPlacement.EquallySpacedRectSide\",\"uuid\":\"c7c95c77-bae3-47b7-a54f-9afc9f4e7b60\"}]},\"type\":\"ConnectorPlacement.EquallySpacedConnector\",\"uuid\":\"47487c21-2009-4dc3-9515-f1b42d882620\"}],\"packageUris\":[\"http://schema.mathworks.com/mf0/Connector/R2020b\"],\"version\":\"1.0\"}"
  Rotation3 : Subsystem  Commented=on
      settings: PortSchema="{\"entries\":[{\"content\":{\"sides\":[{\"content\":{\"connectorIds\":[\"In1\"]},\"type\":\"ConnectorPlacement.EquallySpacedRectSide\",\"uuid\":\"b989bfd3-647b-468d-a24b-67c5817c2fb9\"},{\"content\":{\"connectorIds\":[\"Out1\"],\"side\":\"RIGHT\"},\"type\":\"ConnectorPlacement.EquallySpacedRectSide\",\"uuid\":\"15839450-c6b9-4b4c-b490-793a0225ad70\"},{\"content\":{\"connectorIds\":[\"In2\"],\"side\":\"TOP\"},\"type\":\"ConnectorPlacement.EquallySpacedRectSide\",\"uuid\":\"69a0ff69-1754-49ce-bc12-3d58954b90b5\"},{\"content\":{\"connectorIds\":[\"Out2\"],\"side\":\"BOTTOM\"},\"type\":\"ConnectorPlacement.EquallySpacedRectSide\",\"uuid\":\"c7c95c77-bae3-47b7-a54f-9afc9f4e7b60\"}]},\"type\":\"ConnectorPlacement.EquallySpacedConnector\",\"uuid\":\"47487c21-2009-4dc3-9515-f1b42d882620\"}],\"packageUris\":[\"http://schema.mathworks.com/mf0/Connector/R2020b\"],\"version\":\"1.0\"}"
  Rotation30 : Subsystem  Commented=on
      settings: PortSchema="{\"entries\":[{\"content\":{\"sides\":[{\"content\":{\"connectorIds\":[\"Out3\",\"Out4\",\"In1\"]},\"type\":\"ConnectorPlacement.EquallySpacedRectSide\",\"uuid\":\"b989bfd3-647b-468d-a24b-67c5817c2fb9\"},{\"content\":{\"connectorIds\":[\"Out1\"],\"side\":\"RIGHT\"},\"type\":\"ConnectorPlacement.EquallySpacedRectSide\",\"uuid\":\"15839450-c6b9-4b4c-b490-793a0225ad70\"},{\"content\":{\"connectorIds\":[\"In2\"],\"side\":\"TOP\"},\"type\":\"ConnectorPlacement.EquallySpacedRectSide\",\"uuid\":\"69a0ff69-1754-49ce-bc12-3d58954b90b5\"},{\"content\":{\"connectorIds\":[\"Out2\"],\"side\":\"BOTTOM\"},\"type\":\"ConnectorPlacement.EquallySpacedRectSide\",\"uuid\":\"c7c95c77-bae3-47b7-a54f-9afc9f4e7b60\"}]},\"type\":\"ConnectorPlacement.EquallySpacedConnector\",\"uuid\":\"47487c21-2009-4dc3-9515-f1b42d882620\"}],\"packageUris\":[\"http://schema.mathworks.com/mf0/Connector/R2020b\"],\"version\":\"1.0\"}"
  Rotation31 : Subsystem  Commented=on
      settings: PortSchema="{\"entries\":[{\"content\":{\"sides\":[{\"content\":{\"connectorIds\":[\"Out3\",\"Out4\",\"In1\"]},\"type\":\"ConnectorPlacement.EquallySpacedRectSide\",\"uuid\":\"b989bfd3-647b-468d-a24b-67c5817c2fb9\"},{\"content\":{\"connectorIds\":[\"Out1\"],\"side\":\"RIGHT\"},\"type\":\"ConnectorPlacement.EquallySpacedRectSide\",\"uuid\":\"15839450-c6b9-4b4c-b490-793a0225ad70\"},{\"content\":{\"connectorIds\":[\"In2\"],\"side\":\"TOP\"},\"type\":\"ConnectorPlacement.EquallySpacedRectSide\",\"uuid\":\"69a0ff69-1754-49ce-bc12-3d58954b90b5\"},{\"content\":{\"connectorIds\":[\"Out2\"],\"side\":\"BOTTOM\"},\"type\":\"ConnectorPlacement.EquallySpacedRectSide\",\"uuid\":\"c7c95c77-bae3-47b7-a54f-9afc9f4e7b60\"}]},\"type\":\"ConnectorPlacement.EquallySpacedConnector\",\"uuid\":\"47487c21-2009-4dc3-9515-f1b42d882620\"}],\"packageUris\":[\"http://schema.mathworks.com/mf0/Connector/R2020b\"],\"version\":\"1.0\"}"
  Rotation32 : Subsystem  Commented=on
      settings: PortSchema="{\"entries\":[{\"content\":{\"sides\":[{\"content\":{\"connectorIds\":[\"Out3\",\"Out4\",\"In1\"]},\"type\":\"ConnectorPlacement.EquallySpacedRectSide\",\"uuid\":\"b989bfd3-647b-468d-a24b-67c5817c2fb9\"},{\"content\":{\"connectorIds\":[\"Out1\"],\"side\":\"RIGHT\"},\"type\":\"ConnectorPlacement.EquallySpacedRectSide\",\"uuid\":\"15839450-c6b9-4b4c-b490-793a0225ad70\"},{\"content\":{\"connectorIds\":[\"In2\"],\"side\":\"TOP\"},\"type\":\"ConnectorPlacement.EquallySpacedRectSide\",\"uuid\":\"69a0ff69-1754-49ce-bc12-3d58954b90b5\"},{\"content\":{\"connectorIds\":[\"Out2\"],\"side\":\"BOTTOM\"},\"type\":\"ConnectorPlacement.EquallySpacedRectSide\",\"uuid\":\"c7c95c77-bae3-47b7-a54f-9afc9f4e7b60\"}]},\"type\":\"ConnectorPlacement.EquallySpacedConnector\",\"uuid\":\"47487c21-2009-4dc3-9515-f1b42d882620\"}],\"packageUris\":[\"http://schema.mathworks.com/mf0/Connector/R2020b\"],\"version\":\"1.0\"}"
  Rotation33 : Subsystem  Commented=on
      settings: PortSchema="{\"entries\":[{\"content\":{\"sides\":[{\"content\":{\"connectorIds\":[\"Out3\",\"Out4\",\"In1\"]},\"type\":\"ConnectorPlacement.EquallySpacedRectSide\",\"uuid\":\"b989bfd3-647b-468d-a24b-67c5817c2fb9\"},{\"content\":{\"connectorIds\":[\"Out1\"],\"side\":\"RIGHT\"},\"type\":\"ConnectorPlacement.EquallySpacedRectSide\",\"uuid\":\"15839450-c6b9-4b4c-b490-793a0225ad70\"},{\"content\":{\"connectorIds\":[\"In2\"],\"side\":\"TOP\"},\"type\":\"ConnectorPlacement.EquallySpacedRectSide\",\"uuid\":\"69a0ff69-1754-49ce-bc12-3d58954b90b5\"},{\"content\":{\"connectorIds\":[\"Out2\"],\"side\":\"BOTTOM\"},\"type\":\"ConnectorPlacement.EquallySpacedRectSide\",\"uuid\":\"c7c95c77-bae3-47b7-a54f-9afc9f4e7b60\"}]},\"type\":\"ConnectorPlacement.EquallySpacedConnector\",\"uuid\":\"47487c21-2009-4dc3-9515-f1b42d882620\"}],\"packageUris\":[\"http://schema.mathworks.com/mf0/Connector/R2020b\"],\"version\":\"1.0\"}"
  Rotation34 : Subsystem
      settings: PortSchema="{\"entries\":[{\"content\":{\"sides\":[{\"content\":{\"connectorIds\":[\"In1\",\"In2\"]},\"type\":\"ConnectorPlacement.EquallySpacedRectSide\",\"uuid\":\"b989bfd3-647b-468d-a24b-67c5817c2fb9\"},{\"content\":{\"connectorIds\":[\"Out1\",\"Out2\"],\"side\":\"RIGHT\"},\"type\":\"ConnectorPlacement.EquallySpacedRectSide\",\"uuid\":\"15839450-c6b9-4b4c-b490-793a0225ad70\"},{\"content\":{\"connectorIds\":[\"In3\"],\"side\":\"TOP\"},\"type\":\"ConnectorPlacement.EquallySpacedRectSide\",\"uuid\":\"69a0ff69-1754-49ce-bc12-3d58954b90b5\"},{\"content\":{\"connectorIds\":[\"Out3\",\"Out4\"],\"side\":\"BOTTOM\"},\"type\":\"ConnectorPlacement.EquallySpacedRectSide\",\"uuid\":\"c7c95c77-bae3-47b7-a54f-9afc9f4e7b60\"}]},\"type\":\"ConnectorPlacement.EquallySpacedConnector\",\"uuid\":\"47487c21-2009-4dc3-9515-f1b42d882620\"}],\"packageUris\":[\"http://schema.mathworks.com/mf0/Connector/R2020b\"],\"version\":\"1.0\"}"
  Rotation35 : Subsystem
      settings: PortSchema="{\"entries\":[{\"content\":{\"sides\":[{\"content\":{\"connectorIds\":[\"In1\",\"In2\"]},\"type\":\"ConnectorPlacement.EquallySpacedRectSide\",\"uuid\":\"b989bfd3-647b-468d-a24b-67c5817c2fb9\"},{\"content\":{\"connectorIds\":[\"Out1\",\"Out2\"],\"side\":\"RIGHT\"},\"type\":\"ConnectorPlacement.EquallySpacedRectSide\",\"uuid\":\"15839450-c6b9-4b4c-b490-793a0225ad70\"},{\"content\":{\"connectorIds\":[\"In3\"],\"side\":\"TOP\"},\"type\":\"ConnectorPlacement.EquallySpacedRectSide\",\"uuid\":\"69a0ff69-1754-49ce-bc12-3d58954b90b5\"},{\"content\":{\"connectorIds\":[\"Out3\",\"Out4\"],\"side\":\"BOTTOM\"},\"type\":\"ConnectorPlacement.EquallySpacedRectSide\",\"uuid\":\"c7c95c77-bae3-47b7-a54f-9afc9f4e7b60\"}]},\"type\":\"ConnectorPlacement.EquallySpacedConnector\",\"uuid\":\"47487c21-2009-4dc3-9515-f1b42d882620\"}],\"packageUris\":[\"http://schema.mathworks.com/mf0/Connector/R2020b\"],\"version\":\"1.0\"}"
  Rotation36 : Subsystem
      settings: PortSchema="{\"entries\":[{\"content\":{\"sides\":[{\"content\":{\"connectorIds\":[\"In1\",\"Out5\",\"In2\"]},\"type\":\"ConnectorPlacement.EquallySpacedRectSide\",\"uuid\":\"b989bfd3-647b-468d-a24b-67c5817c2fb9\"},{\"content\":{\"connectorIds\":[\"Out1\",\"Out2\"],\"side\":\"RIGHT\"},\"type\":\"ConnectorPlacement.EquallySpacedRectSide\",\"uuid\":\"15839450-c6b9-4b4c-b490-793a0225ad70\"},{\"content\":{\"connectorIds\":[\"In3\"],\"side\":\"TOP\"},\"type\":\"ConnectorPlacement.EquallySpacedRectSide\",\"uuid\":\"69a0ff69-1754-49ce-bc12-3d58954b90b5\"},{\"content\":{\"connectorIds\":[\"Out3\",\"Out4\"],\"side\":\"BOTTOM\"},\"type\":\"ConnectorPlacement.EquallySpacedRectSide\",\"uuid\":\"c7c95c77-bae3-47b7-a54f-9afc9f4e7b60\"}]},\"type\":\"ConnectorPlacement.EquallySpacedConnector\",\"uuid\":\"47487c21-2009-4dc3-9515-f1b42d882620\"}],\"packageUris\":[\"http://schema.mathworks.com/mf0/Connector/R2020b\"],\"version\":\"1.0\"}"
  Rotation37 : Subsystem
      settings: PortSchema="{\"entries\":[{\"content\":{\"sides\":[{\"content\":{\"connectorIds\":[\"In1\",\"Out5\",\"In2\"]},\"type\":\"ConnectorPlacement.EquallySpacedRectSide\",\"uuid\":\"b989bfd3-647b-468d-a24b-67c5817c2fb9\"},{\"content\":{\"connectorIds\":[\"Out1\",\"Out2\"],\"side\":\"RIGHT\"},\"type\":\"ConnectorPlacement.EquallySpacedRectSide\",\"uuid\":\"15839450-c6b9-4b4c-b490-793a0225ad70\"},{\"content\":{\"connectorIds\":[\"In3\"],\"side\":\"TOP\"},\"type\":\"ConnectorPlacement.EquallySpacedRectSide\",\"uuid\":\"69a0ff69-1754-49ce-bc12-3d58954b90b5\"},{\"content\":{\"connectorIds\":[\"Out3\",\"Out4\"],\"side\":\"BOTTOM\"},\"type\":\"ConnectorPlacement.EquallySpacedRectSide\",\"uuid\":\"c7c95c77-bae3-47b7-a54f-9afc9f4e7b60\"}]},\"type\":\"ConnectorPlacement.EquallySpacedConnector\",\"uuid\":\"47487c21-2009-4dc3-9515-f1b42d882620\"}],\"packageUris\":[\"http://schema.mathworks.com/mf0/Connector/R2020b\"],\"version\":\"1.0\"}"
  Rotation38 : Subsystem
      settings: PortSchema="{\"entries\":[{\"content\":{\"sides\":[{\"content\":{\"connectorIds\":[\"In1\",\"Out5\",\"In2\"]},\"type\":\"ConnectorPlacement.EquallySpacedRectSide\",\"uuid\":\"b989bfd3-647b-468d-a24b-67c5817c2fb9\"},{\"content\":{\"connectorIds\":[\"Out1\",\"Out2\"],\"side\":\"RIGHT\"},\"type\":\"ConnectorPlacement.EquallySpacedRectSide\",\"uuid\":\"15839450-c6b9-4b4c-b490-793a0225ad70\"},{\"content\":{\"connectorIds\":[\"In3\"],\"side\":\"TOP\"},\"type\":\"ConnectorPlacement.EquallySpacedRectSide\",\"uuid\":\"69a0ff69-1754-49ce-bc12-3d58954b90b5\"},{\"content\":{\"connectorIds\":[\"Out3\",\"Out4\"],\"side\":\"BOTTOM\"},\"type\":\"ConnectorPlacement.EquallySpacedRectSide\",\"uuid\":\"c7c95c77-bae3-47b7-a54f-9afc9f4e7b60\"}]},\"type\":\"ConnectorPlacement.EquallySpacedConnector\",\"uuid\":\"47487c21-2009-4dc3-9515-f1b42d882620\"}],\"packageUris\":[\"http://schema.mathworks.com/mf0/Connector/R2020b\"],\"version\":\"1.0\"}"
  Rotation39 : Subsystem
      settings: PortSchema="{\"entries\":[{\"content\":{\"sides\":[{\"content\":{\"connectorIds\":[\"In1\",\"Out5\",\"In2\"]},\"type\":\"ConnectorPlacement.EquallySpacedRectSide\",\"uuid\":\"b989bfd3-647b-468d-a24b-67c5817c2fb9\"},{\"content\":{\"connectorIds\":[\"Out1\",\"Out2\"],\"side\":\"RIGHT\"},\"type\":\"ConnectorPlacement.EquallySpacedRectSide\",\"uuid\":\"15839450-c6b9-4b4c-b490-793a0225ad70\"},{\"content\":{\"connectorIds\":[\"In3\"],\"side\":\"TOP\"},\"type\":\"ConnectorPlacement.EquallySpacedRectSide\",\"uuid\":\"69a0ff69-1754-49ce-bc12-3d58954b90b5\"},{\"content\":{\"connectorIds\":[\"Out3\",\"Out4\"],\"side\":\"BOTTOM\"},\"type\":\"ConnectorPlacement.EquallySpacedRectSide\",\"uuid\":\"c7c95c77-bae3-47b7-a54f-9afc9f4e7b60\"}]},\"type\":\"ConnectorPlacement.EquallySpacedConnector\",\"uuid\":\"47487c21-2009-4dc3-9515-f1b42d882620\"}],\"packageUris\":[\"http://schema.mathworks.com/mf0/Connector/R2020b\"],\"version\":\"1.0\"}"
  Rotation4 : Subsystem  Commented=on
      settings: PortSchema="{\"entries\":[{\"content\":{\"sides\":[{\"content\":{\"connectorIds\":[\"In1\"]},\"type\":\"ConnectorPlacement.EquallySpacedRectSide\",\"uuid\":\"b989bfd3-647b-468d-a24b-67c5817c2fb9\"},{\"content\":{\"connectorIds\":[\"Out1\"],\"side\":\"RIGHT\"},\"type\":\"ConnectorPlacement.EquallySpacedRectSide\",\"uuid\":\"15839450-c6b9-4b4c-b490-793a0225ad70\"},{\"content\":{\"connectorIds\":[\"In2\"],\"side\":\"TOP\"},\"type\":\"ConnectorPlacement.EquallySpacedRectSide\",\"uuid\":\"69a0ff69-1754-49ce-bc12-3d58954b90b5\"},{\"content\":{\"connectorIds\":[\"Out2\"],\"side\":\"BOTTOM\"},\"type\":\"ConnectorPlacement.EquallySpacedRectSide\",\"uuid\":\"c7c95c77-bae3-47b7-a54f-9afc9f4e7b60\"}]},\"type\":\"ConnectorPlacement.EquallySpacedConnector\",\"uuid\":\"47487c21-2009-4dc3-9515-f1b42d882620\"}],\"packageUris\":[\"http://schema.mathworks.com/mf0/Connector/R2020b\"],\"version\":\"1.0\"}"
  Rotation40 : Subsystem
      settings: PortSchema="{\"entries\":[{\"content\":{\"sides\":[{\"content\":{\"connectorIds\":[\"In1\",\"Out5\",\"In2\"]},\"type\":\"ConnectorPlacement.EquallySpacedRectSide\",\"uuid\":\"b989bfd3-647b-468d-a24b-67c5817c2fb9\"},{\"content\":{\"connectorIds\":[\"Out1\",\"Out2\"],\"side\":\"RIGHT\"},\"type\":\"ConnectorPlacement.EquallySpacedRectSide\",\"uuid\":\"15839450-c6b9-4b4c-b490-793a0225ad70\"},{\"content\":{\"connectorIds\":[\"In3\"],\"side\":\"TOP\"},\"type\":\"ConnectorPlacement.EquallySpacedRectSide\",\"uuid\":\"69a0ff69-1754-49ce-bc12-3d58954b90b5\"},{\"content\":{\"connectorIds\":[\"Out3\",\"Out4\"],\"side\":\"BOTTOM\"},\"type\":\"ConnectorPlacement.EquallySpacedRectSide\",\"uuid\":\"c7c95c77-bae3-47b7-a54f-9afc9f4e7b60\"}]},\"type\":\"ConnectorPlacement.EquallySpacedConnector\",\"uuid\":\"47487c21-2009-4dc3-9515-f1b42d882620\"}],\"packageUris\":[\"http://schema.mathworks.com/mf0/Connector/R2020b\"],\"version\":\"1.0\"}"
  Rotation41 : Subsystem
      settings: PortSchema="{\"entries\":[{\"content\":{\"sides\":[{\"content\":{\"connectorIds\":[\"In1\",\"Out5\",\"In2\"]},\"type\":\"ConnectorPlacement.EquallySpacedRectSide\",\"uuid\":\"b989bfd3-647b-468d-a24b-67c5817c2fb9\"},{\"content\":{\"connectorIds\":[\"Out1\",\"Out2\"],\"side\":\"RIGHT\"},\"type\":\"ConnectorPlacement.EquallySpacedRectSide\",\"uuid\":\"15839450-c6b9-4b4c-b490-793a0225ad70\"},{\"content\":{\"connectorIds\":[\"In3\"],\"side\":\"TOP\"},\"type\":\"ConnectorPlacement.EquallySpacedRectSide\",\"uuid\":\"69a0ff69-1754-49ce-bc12-3d58954b90b5\"},{\"content\":{\"connectorIds\":[\"Out3\",\"Out4\"],\"side\":\"BOTTOM\"},\"type\":\"ConnectorPlacement.EquallySpacedRectSide\",\"uuid\":\"c7c95c77-bae3-47b7-a54f-9afc9f4e7b60\"}]},\"type\":\"ConnectorPlacement.EquallySpacedConnector\",\"uuid\":\"47487c21-2009-4dc3-9515-f1b42d882620\"}],\"packageUris\":[\"http://schema.mathworks.com/mf0/Connector/R2020b\"],\"version\":\"1.0\"}"
  Rotation42 : Subsystem
      settings: PortSchema="{\"entries\":[{\"content\":{\"sides\":[{\"content\":{\"connectorIds\":[\"In1\",\"Out5\",\"In2\"]},\"type\":\"ConnectorPlacement.EquallySpacedRectSide\",\"uuid\":\"b989bfd3-647b-468d-a24b-67c5817c2fb9\"},{\"content\":{\"connectorIds\":[\"Out1\",\"Out2\"],\"side\":\"RIGHT\"},\"type\":\"ConnectorPlacement.EquallySpacedRectSide\",\"uuid\":\"15839450-c6b9-4b4c-b490-793a0225ad70\"},{\"content\":{\"connectorIds\":[\"In3\"],\"side\":\"TOP\"},\"type\":\"ConnectorPlacement.EquallySpacedRectSide\",\"uuid\":\"69a0ff69-1754-49ce-bc12-3d58954b90b5\"},{\"content\":{\"connectorIds\":[\"Out3\",\"Out4\"],\"side\":\"BOTTOM\"},\"type\":\"ConnectorPlacement.EquallySpacedRectSide\",\"uuid\":\"c7c95c77-bae3-47b7-a54f-9afc9f4e7b60\"}]},\"type\":\"ConnectorPlacement.EquallySpacedConnector\",\"uuid\":\"47487c21-2009-4dc3-9515-f1b42d882620\"}],\"packageUris\":[\"http://schema.mathworks.com/mf0/Connector/R2020b\"],\"version\":\"1.0\"}"
  Rotation43 : Subsystem
      settings: PortSchema="{\"entries\":[{\"content\":{\"sides\":[{\"content\":{\"connectorIds\":[\"In1\",\"Out5\",\"In2\"]},\"type\":\"ConnectorPlacement.EquallySpacedRectSide\",\"uuid\":\"b989bfd3-647b-468d-a24b-67c5817c2fb9\"},{\"content\":{\"connectorIds\":[\"Out1\",\"Out2\"],\"side\":\"RIGHT\"},\"type\":\"ConnectorPlacement.EquallySpacedRectSide\",\"uuid\":\"15839450-c6b9-4b4c-b490-793a0225ad70\"},{\"content\":{\"connectorIds\":[\"In3\"],\"side\":\"TOP\"},\"type\":\"ConnectorPlacement.EquallySpacedRectSide\",\"uuid\":\"69a0ff69-1754-49ce-bc12-3d58954b90b5\"},{\"content\":{\"connectorIds\":[\"Out3\",\"Out4\"],\"side\":\"BOTTOM\"},\"type\":\"ConnectorPlacement.EquallySpacedRectSide\",\"uuid\":\"c7c95c77-bae3-47b7-a54f-9afc9f4e7b60\"}]},\"type\":\"ConnectorPlacement.EquallySpacedConnector\",\"uuid\":\"47487c21-2009-4dc3-9515-f1b42d882620\"}],\"packageUris\":[\"http://schema.mathworks.com/mf0/Connector/R2020b\"],\"version\":\"1.0\"}"
  Rotation44 : Subsystem
      settings: PortSchema="{\"entries\":[{\"content\":{\"sides\":[{\"content\":{\"connectorIds\":[\"In1\",\"Out5\",\"In2\"]},\"type\":\"ConnectorPlacement.EquallySpacedRectSide\",\"uuid\":\"b989bfd3-647b-468d-a24b-67c5817c2fb9\"},{\"content\":{\"connectorIds\":[\"Out1\",\"Out2\"],\"side\":\"RIGHT\"},\"type\":\"ConnectorPlacement.EquallySpacedRectSide\",\"uuid\":\"15839450-c6b9-4b4c-b490-793a0225ad70\"},{\"content\":{\"connectorIds\":[\"In3\"],\"side\":\"TOP\"},\"type\":\"ConnectorPlacement.EquallySpacedRectSide\",\"uuid\":\"69a0ff69-1754-49ce-bc12-3d58954b90b5\"},{\"content\":{\"connectorIds\":[\"Out3\",\"Out4\"],\"side\":\"BOTTOM\"},\"type\":\"ConnectorPlacement.EquallySpacedRectSide\",\"uuid\":\"c7c95c77-bae3-47b7-a54f-9afc9f4e7b60\"}]},\"type\":\"ConnectorPlacement.EquallySpacedConnector\",\"uuid\":\"47487c21-2009-4dc3-9515-f1b42d882620\"}],\"packageUris\":[\"http://schema.mathworks.com/mf0/Connector/R2020b\"],\"version\":\"1.0\"}"
  Rotation45 : Subsystem
      settings: PortSchema="{\"entries\":[{\"content\":{\"sides\":[{\"content\":{\"connectorIds\":[\"In1\",\"Out5\",\"In2\"]},\"type\":\"ConnectorPlacement.EquallySpacedRectSide\",\"uuid\":\"b989bfd3-647b-468d-a24b-67c5817c2fb9\"},{\"content\":{\"connectorIds\":[\"Out1\",\"Out2\"],\"side\":\"RIGHT\"},\"type\":\"ConnectorPlacement.EquallySpacedRectSide\",\"uuid\":\"15839450-c6b9-4b4c-b490-793a0225ad70\"},{\"content\":{\"connectorIds\":[\"In3\"],\"side\":\"TOP\"},\"type\":\"ConnectorPlacement.EquallySpacedRectSide\",\"uuid\":\"69a0ff69-1754-49ce-bc12-3d58954b90b5\"},{\"content\":{\"connectorIds\":[\"Out3\",\"Out4\"],\"side\":\"BOTTOM\"},\"type\":\"ConnectorPlacement.EquallySpacedRectSide\",\"uuid\":\"c7c95c77-bae3-47b7-a54f-9afc9f4e7b60\"}]},\"type\":\"ConnectorPlacement.EquallySpacedConnector\",\"uuid\":\"47487c21-2009-4dc3-9515-f1b42d882620\"}],\"packageUris\":[\"http://schema.mathworks.com/mf0/Connector/R2020b\"],\"version\":\"1.0\"}"
  Rotation46 : Subsystem
      settings: PortSchema="{\"entries\":[{\"content\":{\"sides\":[{\"content\":{\"connectorIds\":[\"In1\",\"Out5\",\"In2\"]},\"type\":\"ConnectorPlacement.EquallySpacedRectSide\",\"uuid\":\"b989bfd3-647b-468d-a24b-67c5817c2fb9\"},{\"content\":{\"connectorIds\":[\"Out1\",\"Out2\"],\"side\":\"RIGHT\"},\"type\":\"ConnectorPlacement.EquallySpacedRectSide\",\"uuid\":\"15839450-c6b9-4b4c-b490-793a0225ad70\"},{\"content\":{\"connectorIds\":[\"In3\"],\"side\":\"TOP\"},\"type\":\"ConnectorPlacement.EquallySpacedRectSide\",\"uuid\":\"69a0ff69-1754-49ce-bc12-3d58954b90b5\"},{\"content\":{\"connectorIds\":[\"Out3\",\"Out4\"],\"side\":\"BOTTOM\"},\"type\":\"ConnectorPlacement.EquallySpacedRectSide\",\"uuid\":\"c7c95c77-bae3-47b7-a54f-9afc9f4e7b60\"}]},\"type\":\"ConnectorPlacement.EquallySpacedConnector\",\"uuid\":\"47487c21-2009-4dc3-9515-f1b42d882620\"}],\"packageUris\":[\"http://schema.mathworks.com/mf0/Connector/R2020b\"],\"version\":\"1.0\"}"
  Rotation47 : Subsystem
      settings: PortSchema="{\"entries\":[{\"content\":{\"sides\":[{\"content\":{\"connectorIds\":[\"In1\",\"Out5\",\"In2\"]},\"type\":\"ConnectorPlacement.EquallySpacedRectSide\",\"uuid\":\"b989bfd3-647b-468d-a24b-67c5817c2fb9\"},{\"content\":{\"connectorIds\":[\"Out1\",\"Out2\"],\"side\":\"RIGHT\"},\"type\":\"ConnectorPlacement.EquallySpacedRectSide\",\"uuid\":\"15839450-c6b9-4b4c-b490-793a0225ad70\"},{\"content\":{\"connectorIds\":[\"In3\"],\"side\":\"TOP\"},\"type\":\"ConnectorPlacement.EquallySpacedRectSide\",\"uuid\":\"69a0ff69-1754-49ce-bc12-3d58954b90b5\"},{\"content\":{\"connectorIds\":[\"Out3\",\"Out4\"],\"side\":\"BOTTOM\"},\"type\":\"ConnectorPlacement.EquallySpacedRectSide\",\"uuid\":\"c7c95c77-bae3-47b7-a54f-9afc9f4e7b60\"}]},\"type\":\"ConnectorPlacement.EquallySpacedConnector\",\"uuid\":\"47487c21-2009-4dc3-9515-f1b42d882620\"}],\"packageUris\":[\"http://schema.mathworks.com/mf0/Connector/R2020b\"],\"version\":\"1.0\"}"
  Rotation48 : Subsystem
      settings: PortSchema="{\"entries\":[{\"content\":{\"sides\":[{\"content\":{\"connectorIds\":[\"In1\",\"Out5\",\"In2\"]},\"type\":\"ConnectorPlacement.EquallySpacedRectSide\",\"uuid\":\"b989bfd3-647b-468d-a24b-67c5817c2fb9\"},{\"content\":{\"connectorIds\":[\"Out1\",\"Out2\"],\"side\":\"RIGHT\"},\"type\":\"ConnectorPlacement.EquallySpacedRectSide\",\"uuid\":\"15839450-c6b9-4b4c-b490-793a0225ad70\"},{\"content\":{\"connectorIds\":[\"In3\"],\"side\":\"TOP\"},\"type\":\"ConnectorPlacement.EquallySpacedRectSide\",\"uuid\":\"69a0ff69-1754-49ce-bc12-3d58954b90b5\"},{\"content\":{\"connectorIds\":[\"Out3\",\"Out4\"],\"side\":\"BOTTOM\"},\"type\":\"ConnectorPlacement.EquallySpacedRectSide\",\"uuid\":\"c7c95c77-bae3-47b7-a54f-9afc9f4e7b60\"}]},\"type\":\"ConnectorPlacement.EquallySpacedConnector\",\"uuid\":\"47487c21-2009-4dc3-9515-f1b42d882620\"}],\"packageUris\":[\"http://schema.mathworks.com/mf0/Connector/R2020b\"],\"version\":\"1.0\"}"
  Rotation49 : Subsystem
      settings: PortSchema="{\"entries\":[{\"content\":{\"sides\":[{\"content\":{\"connectorIds\":[\"In1\",\"Out5\",\"In2\"]},\"type\":\"ConnectorPlacement.EquallySpacedRectSide\",\"uuid\":\"b989bfd3-647b-468d-a24b-67c5817c2fb9\"},{\"content\":{\"connectorIds\":[\"Out1\",\"Out2\"],\"side\":\"RIGHT\"},\"type\":\"ConnectorPlacement.EquallySpacedRectSide\",\"uuid\":\"15839450-c6b9-4b4c-b490-793a0225ad70\"},{\"content\":{\"connectorIds\":[\"In3\"],\"side\":\"TOP\"},\"type\":\"ConnectorPlacement.EquallySpacedRectSide\",\"uuid\":\"69a0ff69-1754-49ce-bc12-3d58954b90b5\"},{\"content\":{\"connectorIds\":[\"Out3\",\"Out4\"],\"side\":\"BOTTOM\"},\"type\":\"ConnectorPlacement.EquallySpacedRectSide\",\"uuid\":\"c7c95c77-bae3-47b7-a54f-9afc9f4e7b60\"}]},\"type\":\"ConnectorPlacement.EquallySpacedConnector\",\"uuid\":\"47487c21-2009-4dc3-9515-f1b42d882620\"}],\"packageUris\":[\"http://schema.mathworks.com/mf0/Connector/R2020b\"],\"version\":\"1.0\"}"
  Rotation5 : Subsystem  Commented=on
      settings: PortSchema="{\"entries\":[{\"content\":{\"sides\":[{\"content\":{\"connectorIds\":[\"In1\"]},\"type\":\"ConnectorPlacement.EquallySpacedRectSide\",\"uuid\":\"b989bfd3-647b-468d-a24b-67c5817c2fb9\"},{\"content\":{\"connectorIds\":[\"Out1\"],\"side\":\"RIGHT\"},\"type\":\"ConnectorPlacement.EquallySpacedRectSide\",\"uuid\":\"15839450-c6b9-4b4c-b490-793a0225ad70\"},{\"content\":{\"connectorIds\":[\"In2\"],\"side\":\"TOP\"},\"type\":\"ConnectorPlacement.EquallySpacedRectSide\",\"uuid\":\"69a0ff69-1754-49ce-bc12-3d58954b90b5\"},{\"content\":{\"connectorIds\":[\"Out2\"],\"side\":\"BOTTOM\"},\"type\":\"ConnectorPlacement.EquallySpacedRectSide\",\"uuid\":\"c7c95c77-bae3-47b7-a54f-9afc9f4e7b60\"}]},\"type\":\"ConnectorPlacement.EquallySpacedConnector\",\"uuid\":\"47487c21-2009-4dc3-9515-f1b42d882620\"}],\"packageUris\":[\"http://schema.mathworks.com/mf0/Connector/R2020b\"],\"version\":\"1.0\"}"
  Rotation50 : Subsystem
      settings: PortSchema="{\"entries\":[{\"content\":{\"sides\":[{\"content\":{\"connectorIds\":[\"In1\",\"Out5\",\"In2\"]},\"type\":\"ConnectorPlacement.EquallySpacedRectSide\",\"uuid\":\"b989bfd3-647b-468d-a24b-67c5817c2fb9\"},{\"content\":{\"connectorIds\":[\"Out1\",\"Out2\"],\"side\":\"RIGHT\"},\"type\":\"ConnectorPlacement.EquallySpacedRectSide\",\"uuid\":\"15839450-c6b9-4b4c-b490-793a0225ad70\"},{\"content\":{\"connectorIds\":[\"In3\"],\"side\":\"TOP\"},\"type\":\"ConnectorPlacement.EquallySpacedRectSide\",\"uuid\":\"69a0ff69-1754-49ce-bc12-3d58954b90b5\"},{\"content\":{\"connectorIds\":[\"Out3\",\"Out4\"],\"side\":\"BOTTOM\"},\"type\":\"ConnectorPlacement.EquallySpacedRectSide\",\"uuid\":\"c7c95c77-bae3-47b7-a54f-9afc9f4e7b60\"}]},\"type\":\"ConnectorPlacement.EquallySpacedConnector\",\"uuid\":\"47487c21-2009-4dc3-9515-f1b42d882620\"}],\"packageUris\":[\"http://schema.mathworks.com/mf0/Connector/R2020b\"],\"version\":\"1.0\"}"
  Rotation51 : Subsystem
      settings: PortSchema="{\"entries\":[{\"content\":{\"sides\":[{\"content\":{\"connectorIds\":[\"In1\",\"Out5\",\"In2\"]},\"type\":\"ConnectorPlacement.EquallySpacedRectSide\",\"uuid\":\"b989bfd3-647b-468d-a24b-67c5817c2fb9\"},{\"content\":{\"connectorIds\":[\"Out1\",\"Out2\"],\"side\":\"RIGHT\"},\"type\":\"ConnectorPlacement.EquallySpacedRectSide\",\"uuid\":\"15839450-c6b9-4b4c-b490-793a0225ad70\"},{\"content\":{\"connectorIds\":[\"In3\"],\"side\":\"TOP\"},\"type\":\"ConnectorPlacement.EquallySpacedRectSide\",\"uuid\":\"69a0ff69-1754-49ce-bc12-3d58954b90b5\"},{\"content\":{\"connectorIds\":[\"Out3\",\"Out4\"],\"side\":\"BOTTOM\"},\"type\":\"ConnectorPlacement.EquallySpacedRectSide\",\"uuid\":\"c7c95c77-bae3-47b7-a54f-9afc9f4e7b60\"}]},\"type\":\"ConnectorPlacement.EquallySpacedConnector\",\"uuid\":\"47487c21-2009-4dc3-9515-f1b42d882620\"}],\"packageUris\":[\"http://schema.mathworks.com/mf0/Connector/R2020b\"],\"version\":\"1.0\"}"
  Rotation6 : Subsystem  Commented=on
      settings: PortSchema="{\"entries\":[{\"content\":{\"sides\":[{\"content\":{\"connectorIds\":[\"In1\"]},\"type\":\"ConnectorPlacement.EquallySpacedRectSide\",\"uuid\":\"b989bfd3-647b-468d-a24b-67c5817c2fb9\"},{\"content\":{\"connectorIds\":[\"Out1\"],\"side\":\"RIGHT\"},\"type\":\"ConnectorPlacement.EquallySpacedRectSide\",\"uuid\":\"15839450-c6b9-4b4c-b490-793a0225ad70\"},{\"content\":{\"connectorIds\":[\"In2\"],\"side\":\"TOP\"},\"type\":\"ConnectorPlacement.EquallySpacedRectSide\",\"uuid\":\"69a0ff69-1754-49ce-bc12-3d58954b90b5\"},{\"content\":{\"connectorIds\":[\"Out2\"],\"side\":\"BOTTOM\"},\"type\":\"ConnectorPlacement.EquallySpacedRectSide\",\"uuid\":\"c7c95c77-bae3-47b7-a54f-9afc9f4e7b60\"}]},\"type\":\"ConnectorPlacement.EquallySpacedConnector\",\"uuid\":\"47487c21-2009-4dc3-9515-f1b42d882620\"}],\"packageUris\":[\"http://schema.mathworks.com/mf0/Connector/R2020b\"],\"version\":\"1.0\"}"
  Rotation7 : Subsystem  Commented=on
      settings: PortSchema="{\"entries\":[{\"content\":{\"sides\":[{\"content\":{\"connectorIds\":[\"In1\"]},\"type\":\"ConnectorPlacement.EquallySpacedRectSide\",\"uuid\":\"b989bfd3-647b-468d-a24b-67c5817c2fb9\"},{\"content\":{\"connectorIds\":[\"Out1\"],\"side\":\"RIGHT\"},\"type\":\"ConnectorPlacement.EquallySpacedRectSide\",\"uuid\":\"15839450-c6b9-4b4c-b490-793a0225ad70\"},{\"content\":{\"connectorIds\":[\"In2\"],\"side\":\"TOP\"},\"type\":\"ConnectorPlacement.EquallySpacedRectSide\",\"uuid\":\"69a0ff69-1754-49ce-bc12-3d58954b90b5\"},{\"content\":{\"connectorIds\":[\"Out2\"],\"side\":\"BOTTOM\"},\"type\":\"ConnectorPlacement.EquallySpacedRectSide\",\"uuid\":\"c7c95c77-bae3-47b7-a54f-9afc9f4e7b60\"}]},\"type\":\"ConnectorPlacement.EquallySpacedConnector\",\"uuid\":\"47487c21-2009-4dc3-9515-f1b42d882620\"}],\"packageUris\":[\"http://schema.mathworks.com/mf0/Connector/R2020b\"],\"version\":\"1.0\"}"
  Rotation8 : Subsystem  Commented=on
      settings: PortSchema="{\"entries\":[{\"content\":{\"sides\":[{\"content\":{\"connectorIds\":[\"In1\"]},\"type\":\"ConnectorPlacement.EquallySpacedRectSide\",\"uuid\":\"b989bfd3-647b-468d-a24b-67c5817c2fb9\"},{\"content\":{\"connectorIds\":[\"Out1\"],\"side\":\"RIGHT\"},\"type\":\"ConnectorPlacement.EquallySpacedRectSide\",\"uuid\":\"15839450-c6b9-4b4c-b490-793a0225ad70\"},{\"content\":{\"connectorIds\":[\"In2\"],\"side\":\"TOP\"},\"type\":\"ConnectorPlacement.EquallySpacedRectSide\",\"uuid\":\"69a0ff69-1754-49ce-bc12-3d58954b90b5\"},{\"content\":{\"connectorIds\":[\"Out2\"],\"side\":\"BOTTOM\"},\"type\":\"ConnectorPlacement.EquallySpacedRectSide\",\"uuid\":\"c7c95c77-bae3-47b7-a54f-9afc9f4e7b60\"}]},\"type\":\"ConnectorPlacement.EquallySpacedConnector\",\"uuid\":\"47487c21-2009-4dc3-9515-f1b42d882620\"}],\"packageUris\":[\"http://schema.mathworks.com/mf0/Connector/R2020b\"],\"version\":\"1.0\"}"
  Rotation9 : Subsystem  Commented=on
      settings: PortSchema="{\"entries\":[{\"content\":{\"sides\":[{\"content\":{\"connectorIds\":[\"In1\"]},\"type\":\"ConnectorPlacement.EquallySpacedRectSide\",\"uuid\":\"b989bfd3-647b-468d-a24b-67c5817c2fb9\"},{\"content\":{\"connectorIds\":[\"Out1\"],\"side\":\"RIGHT\"},\"type\":\"ConnectorPlacement.EquallySpacedRectSide\",\"uuid\":\"15839450-c6b9-4b4c-b490-793a0225ad70\"},{\"content\":{\"connectorIds\":[\"In2\"],\"side\":\"TOP\"},\"type\":\"ConnectorPlacement.EquallySpacedRectSide\",\"uuid\":\"69a0ff69-1754-49ce-bc12-3d58954b90b5\"},{\"content\":{\"connectorIds\":[\"Out2\"],\"side\":\"BOTTOM\"},\"type\":\"ConnectorPlacement.EquallySpacedRectSide\",\"uuid\":\"c7c95c77-bae3-47b7-a54f-9afc9f4e7b60\"}]},\"type\":\"ConnectorPlacement.EquallySpacedConnector\",\"uuid\":\"47487c21-2009-4dc3-9515-f1b42d882620\"}],\"packageUris\":[\"http://schema.mathworks.com/mf0/Connector/R2020b\"],\"version\":\"1.0\"}"
  Scope : Scope  Commented=on  NumInputPorts=3
  Scope{1,4..7,9} (6 alike) : Scope  Commented=on  NumInputPorts=2
  Scope{3,8,10,12..38,40..50} (41 alike) : Scope  Commented=on
  Scope11 : Scope  Commented=on  NumInputPorts=3
  Scope2 : Scope  Commented=on  NumInputPorts=3
  Scope{54..75} (22 alike) : Scope
  Terminator{,1..9,11..26,43,46..49,51..54} (35 alike) : Terminator  Commented=on
  Terminator{10,27..42,45} (18 alike) : Terminator
  To Workspace : ToWorkspace  Commented=on  VariableName=simout  SaveFormat=Timeseries  SampleTime=-1
  To Workspace1 : ToWorkspace  Commented=on  VariableName=simout1  SaveFormat=Timeseries  SampleTime=-1
  To Workspace10 : ToWorkspace  Commented=on  VariableName=simout10  SaveFormat=Timeseries  SampleTime=-1
  To Workspace11 : ToWorkspace  Commented=on  VariableName=simout11  SaveFormat=Timeseries  SampleTime=-1
  To Workspace12 : ToWorkspace  VariableName=simout40  SaveFormat=Timeseries  SampleTime=-1
  To Workspace13 : ToWorkspace  Commented=on  VariableName=simout13  SaveFormat=Timeseries  SampleTime=-1
  To Workspace14 : ToWorkspace  Commented=on  VariableName=simout14  SaveFormat=Timeseries  SampleTime=-1
  To Workspace15 : ToWorkspace  Commented=on  VariableName=simout15  SaveFormat=Timeseries  SampleTime=-1
  To Workspace16 : ToWorkspace  Commented=on  VariableName=simout16  SaveFormat=Timeseries  SampleTime=-1
  To Workspace17 : ToWorkspace  Commented=on  VariableName=simout17  SaveFormat=Timeseries  SampleTime=-1
  To Workspace18 : ToWorkspace  Commented=on  VariableName=simout18  SaveFormat=Timeseries  SampleTime=-1
  To Workspace19 : ToWorkspace  Commented=on  VariableName=simout19  SaveFormat=Timeseries  SampleTime=-1
  To Workspace2 : ToWorkspace  Commented=on  VariableName=simout2  SaveFormat=Timeseries  SampleTime=-1
  To Workspace20 : ToWorkspace  VariableName=simout41  SaveFormat=Timeseries  SampleTime=-1
  To Workspace21 : ToWorkspace  VariableName=simout42  SaveFormat=Timeseries  SampleTime=-1
  To Workspace22 : ToWorkspace  VariableName=simout43  SaveFormat=Timeseries  SampleTime=-1
  To Workspace23 : ToWorkspace  VariableName=simout44  SaveFormat=Timeseries  SampleTime=-1
  To Workspace24 : ToWorkspace  Commented=on  VariableName=simout45  SaveFormat=Timeseries  SampleTime=-1
  To Workspace3 : ToWorkspace  Commented=on  VariableName=simout3  SaveFormat=Timeseries  SampleTime=-1
  To Workspace4 : ToWorkspace  Commented=on  VariableName=simout4  SaveFormat=Timeseries  SampleTime=-1
  To Workspace5 : ToWorkspace  Commented=on  VariableName=simout5  SaveFormat=Timeseries  SampleTime=-1
  To Workspace6 : ToWorkspace  Commented=on  VariableName=simout6  SaveFormat=Timeseries  SampleTime=-1
  To Workspace7 : ToWorkspace  Commented=on  VariableName=simout7  SaveFormat=Timeseries  SampleTime=-1
  To Workspace8 : ToWorkspace  Commented=on  VariableName=simout8  SaveFormat=Timeseries  SampleTime=-1
  To Workspace9 : ToWorkspace  Commented=on  VariableName=simout9  SaveFormat=Timeseries  SampleTime=-1
  Vectoring : Subsystem  Commented=on
      settings: PortSchema="{\"entries\":[{\"content\":{\"sides\":[{\"content\":{\"connectorIds\":[]},\"type\":\"ConnectorPlacement.EquallySpacedRectSide\",\"uuid\":\"7f0919a1-928c-4229-a557-ae6b37c0e18a\"},{\"content\":{\"connectorIds\":[\"Out1\"],\"side\":\"RIGHT\"},\"type\":\"ConnectorPlacement.EquallySpacedRectSide\",\"uuid\":\"c3dbff62-2cbb-49e5-a718-27c684f0604c\"},{\"content\":{\"connectorIds\":[\"In1\"],\"side\":\"TOP\"},\"type\":\"ConnectorPlacement.EquallySpacedRectSide\",\"uuid\":\"83a064d4-85ee-4dcc-804e-22587799da9e\"}]},\"type\":\"ConnectorPlacement.EquallySpacedConnector\",\"uuid\":\"6d33be0e-4d36-4c84-a292-f5ef4e252a8e\"}],\"packageUris\":[\"http://schema.mathworks.com/mf0/Connector/R2020b\"],\"version\":\"1.0\"}"
  Vectoring1 : Subsystem  Commented=on
      settings: PortSchema="{\"entries\":[{\"content\":{\"sides\":[{\"content\":{\"connectorIds\":[]},\"type\":\"ConnectorPlacement.EquallySpacedRectSide\",\"uuid\":\"7f0919a1-928c-4229-a557-ae6b37c0e18a\"},{\"content\":{\"connectorIds\":[\"Out1\"],\"side\":\"RIGHT\"},\"type\":\"ConnectorPlacement.EquallySpacedRectSide\",\"uuid\":\"c3dbff62-2cbb-49e5-a718-27c684f0604c\"},{\"content\":{\"connectorIds\":[\"In1\"],\"side\":\"TOP\"},\"type\":\"ConnectorPlacement.EquallySpacedRectSide\",\"uuid\":\"83a064d4-85ee-4dcc-804e-22587799da9e\"}]},\"type\":\"ConnectorPlacement.EquallySpacedConnector\",\"uuid\":\"6d33be0e-4d36-4c84-a292-f5ef4e252a8e\"}],\"packageUris\":[\"http://schema.mathworks.com/mf0/Connector/R2020b\"],\"version\":\"1.0\"}"
  Vectoring10 : Subsystem  Commented=on
      settings: PortSchema="{\"entries\":[{\"content\":{\"sides\":[{\"content\":{\"connectorIds\":[]},\"type\":\"ConnectorPlacement.EquallySpacedRectSide\",\"uuid\":\"7f0919a1-928c-4229-a557-ae6b37c0e18a\"},{\"content\":{\"connectorIds\":[\"Out1\",\"Out2\"],\"side\":\"RIGHT\"},\"type\":\"ConnectorPlacement.EquallySpacedRectSide\",\"uuid\":\"c3dbff62-2cbb-49e5-a718-27c684f0604c\"},{\"content\":{\"connectorIds\":[\"In1\"],\"side\":\"TOP\"},\"type\":\"ConnectorPlacement.EquallySpacedRectSide\",\"uuid\":\"83a064d4-85ee-4dcc-804e-22587799da9e\"}]},\"type\":\"ConnectorPlacement.EquallySpacedConnector\",\"uuid\":\"6d33be0e-4d36-4c84-a292-f5ef4e252a8e\"}],\"packageUris\":[\"http://schema.mathworks.com/mf0/Connector/R2020b\"],\"version\":\"1.0\"}"
  Vectoring11 : Subsystem  Commented=on
      settings: PortSchema="{\"entries\":[{\"content\":{\"sides\":[{\"content\":{\"connectorIds\":[]},\"type\":\"ConnectorPlacement.EquallySpacedRectSide\",\"uuid\":\"7f0919a1-928c-4229-a557-ae6b37c0e18a\"},{\"content\":{\"connectorIds\":[\"Out1\",\"Out2\"],\"side\":\"RIGHT\"},\"type\":\"ConnectorPlacement.EquallySpacedRectSide\",\"uuid\":\"c3dbff62-2cbb-49e5-a718-27c684f0604c\"},{\"content\":{\"connectorIds\":[\"In1\"],\"side\":\"TOP\"},\"type\":\"ConnectorPlacement.EquallySpacedRectSide\",\"uuid\":\"83a064d4-85ee-4dcc-804e-22587799da9e\"}]},\"type\":\"ConnectorPlacement.EquallySpacedConnector\",\"uuid\":\"6d33be0e-4d36-4c84-a292-f5ef4e252a8e\"}],\"packageUris\":[\"http://schema.mathworks.com/mf0/Connector/R2020b\"],\"version\":\"1.0\"}"
  Vectoring12 : Subsystem
      settings: PortSchema="{\"entries\":[{\"content\":{\"sides\":[{\"content\":{\"connectorIds\":[]},\"type\":\"ConnectorPlacement.EquallySpacedRectSide\",\"uuid\":\"7f0919a1-928c-4229-a557-ae6b37c0e18a\"},{\"content\":{\"connectorIds\":[\"Out1\",\"Out2\"],\"side\":\"RIGHT\"},\"type\":\"ConnectorPlacement.EquallySpacedRectSide\",\"uuid\":\"c3dbff62-2cbb-49e5-a718-27c684f0604c\"},{\"content\":{\"connectorIds\":[\"In1\",\"In2\"],\"side\":\"TOP\"},\"type\":\"ConnectorPlacement.EquallySpacedRectSide\",\"uuid\":\"83a064d4-85ee-4dcc-804e-22587799da9e\"},{\"content\":{\"connectorIds\":[\"Out3\"],\"side\":\"BOTTOM\"},\"type\":\"ConnectorPlacement.EquallySpacedRectSide\",\"uuid\":\"eea76909-33f2-4847-bfa0-f6ca22c12ff2\"}]},\"type\":\"ConnectorPlacement.EquallySpacedConnector\",\"uuid\":\"6d33be0e-4d36-4c84-a292-f5ef4e252a8e\"}],\"packageUris\":[\"http://schema.mathworks.com/mf0/Connector/R2020b\"],\"version\":\"1.0\"}"
  Vectoring14 : Subsystem
      settings: PortSchema="{\"entries\":[{\"content\":{\"sides\":[{\"content\":{\"connectorIds\":[]},\"type\":\"ConnectorPlacement.EquallySpacedRectSide\",\"uuid\":\"7f0919a1-928c-4229-a557-ae6b37c0e18a\"},{\"content\":{\"connectorIds\":[\"Out1\",\"Out2\"],\"side\":\"RIGHT\"},\"type\":\"ConnectorPlacement.EquallySpacedRectSide\",\"uuid\":\"c3dbff62-2cbb-49e5-a718-27c684f0604c\"},{\"content\":{\"connectorIds\":[\"In1\",\"In2\"],\"side\":\"TOP\"},\"type\":\"ConnectorPlacement.EquallySpacedRectSide\",\"uuid\":\"83a064d4-85ee-4dcc-804e-22587799da9e\"},{\"content\":{\"connectorIds\":[],\"side\":\"BOTTOM\"},\"type\":\"ConnectorPlacement.EquallySpacedRectSide\",\"uuid\":\"eea76909-33f2-4847-bfa0-f6ca22c12ff2\"}]},\"type\":\"ConnectorPlacement.EquallySpacedConnector\",\"uuid\":\"6d33be0e-4d36-4c84-a292-f5ef4e252a8e\"}],\"packageUris\":[\"http://schema.mathworks.com/mf0/Connector/R2020b\"],\"version\":\"1.0\"}"
  Vectoring15 : Subsystem
      settings: PortSchema="{\"entries\":[{\"content\":{\"sides\":[{\"content\":{\"connectorIds\":[]},\"type\":\"ConnectorPlacement.EquallySpacedRectSide\",\"uuid\":\"7f0919a1-928c-4229-a557-ae6b37c0e18a\"},{\"content\":{\"connectorIds\":[\"Out1\",\"Out2\"],\"side\":\"RIGHT\"},\"type\":\"ConnectorPlacement.EquallySpacedRectSide\",\"uuid\":\"c3dbff62-2cbb-49e5-a718-27c684f0604c\"},{\"content\":{\"connectorIds\":[\"In1\",\"In2\"],\"side\":\"TOP\"},\"type\":\"ConnectorPlacement.EquallySpacedRectSide\",\"uuid\":\"83a064d4-85ee-4dcc-804e-22587799da9e\"},{\"content\":{\"connectorIds\":[\"Out3\"],\"side\":\"BOTTOM\"},\"type\":\"ConnectorPlacement.EquallySpacedRectSide\",\"uuid\":\"eea76909-33f2-4847-bfa0-f6ca22c12ff2\"}]},\"type\":\"ConnectorPlacement.EquallySpacedConnector\",\"uuid\":\"6d33be0e-4d36-4c84-a292-f5ef4e252a8e\"}],\"packageUris\":[\"http://schema.mathworks.com/mf0/Connector/R2020b\"],\"version\":\"1.0\"}"
  Vectoring2 : Subsystem  Commented=on
      settings: PortSchema="{\"entries\":[{\"content\":{\"sides\":[{\"content\":{\"connectorIds\":[]},\"type\":\"ConnectorPlacement.EquallySpacedRectSide\",\"uuid\":\"7f0919a1-928c-4229-a557-ae6b37c0e18a\"},{\"content\":{\"connectorIds\":[\"Out1\"],\"side\":\"RIGHT\"},\"type\":\"ConnectorPlacement.EquallySpacedRectSide\",\"uuid\":\"c3dbff62-2cbb-49e5-a718-27c684f0604c\"},{\"content\":{\"connectorIds\":[\"In1\"],\"side\":\"TOP\"},\"type\":\"ConnectorPlacement.EquallySpacedRectSide\",\"uuid\":\"83a064d4-85ee-4dcc-804e-22587799da9e\"}]},\"type\":\"ConnectorPlacement.EquallySpacedConnector\",\"uuid\":\"6d33be0e-4d36-4c84-a292-f5ef4e252a8e\"}],\"packageUris\":[\"http://schema.mathworks.com/mf0/Connector/R2020b\"],\"version\":\"1.0\"}"
  Vectoring3 : Subsystem  Commented=on
      settings: PortSchema="{\"entries\":[{\"content\":{\"sides\":[{\"content\":{\"connectorIds\":[]},\"type\":\"ConnectorPlacement.EquallySpacedRectSide\",\"uuid\":\"7f0919a1-928c-4229-a557-ae6b37c0e18a\"},{\"content\":{\"connectorIds\":[\"Out1\"],\"side\":\"RIGHT\"},\"type\":\"ConnectorPlacement.EquallySpacedRectSide\",\"uuid\":\"c3dbff62-2cbb-49e5-a718-27c684f0604c\"},{\"content\":{\"connectorIds\":[\"In1\"],\"side\":\"TOP\"},\"type\":\"ConnectorPlacement.EquallySpacedRectSide\",\"uuid\":\"83a064d4-85ee-4dcc-804e-22587799da9e\"}]},\"type\":\"ConnectorPlacement.EquallySpacedConnector\",\"uuid\":\"6d33be0e-4d36-4c84-a292-f5ef4e252a8e\"}],\"packageUris\":[\"http://schema.mathworks.com/mf0/Connector/R2020b\"],\"version\":\"1.0\"}"
  Vectoring4 : Subsystem  Commented=on
      settings: PortSchema="{\"entries\":[{\"content\":{\"sides\":[{\"content\":{\"connectorIds\":[]},\"type\":\"ConnectorPlacement.EquallySpacedRectSide\",\"uuid\":\"7f0919a1-928c-4229-a557-ae6b37c0e18a\"},{\"content\":{\"connectorIds\":[\"Out1\"],\"side\":\"RIGHT\"},\"type\":\"ConnectorPlacement.EquallySpacedRectSide\",\"uuid\":\"c3dbff62-2cbb-49e5-a718-27c684f0604c\"},{\"content\":{\"connectorIds\":[\"In1\"],\"side\":\"TOP\"},\"type\":\"ConnectorPlacement.EquallySpacedRectSide\",\"uuid\":\"83a064d4-85ee-4dcc-804e-22587799da9e\"}]},\"type\":\"ConnectorPlacement.EquallySpacedConnector\",\"uuid\":\"6d33be0e-4d36-4c84-a292-f5ef4e252a8e\"}],\"packageUris\":[\"http://schema.mathworks.com/mf0/Connector/R2020b\"],\"version\":\"1.0\"}"
  Vectoring5 : Subsystem  Commented=on
      settings: PortSchema="{\"entries\":[{\"content\":{\"sides\":[{\"content\":{\"connectorIds\":[]},\"type\":\"ConnectorPlacement.EquallySpacedRectSide\",\"uuid\":\"7f0919a1-928c-4229-a557-ae6b37c0e18a\"},{\"content\":{\"connectorIds\":[\"Out1\"],\"side\":\"RIGHT\"},\"type\":\"ConnectorPlacement.EquallySpacedRectSide\",\"uuid\":\"c3dbff62-2cbb-49e5-a718-27c684f0604c\"},{\"content\":{\"connectorIds\":[\"In1\"],\"side\":\"TOP\"},\"type\":\"ConnectorPlacement.EquallySpacedRectSide\",\"uuid\":\"83a064d4-85ee-4dcc-804e-22587799da9e\"}]},\"type\":\"ConnectorPlacement.EquallySpacedConnector\",\"uuid\":\"6d33be0e-4d36-4c84-a292-f5ef4e252a8e\"}],\"packageUris\":[\"http://schema.mathworks.com/mf0/Connector/R2020b\"],\"version\":\"1.0\"}"
  Vectoring6 : Subsystem  Commented=on
      settings: PortSchema="{\"entries\":[{\"content\":{\"sides\":[{\"content\":{\"connectorIds\":[]},\"type\":\"ConnectorPlacement.EquallySpacedRectSide\",\"uuid\":\"7f0919a1-928c-4229-a557-ae6b37c0e18a\"},{\"content\":{\"connectorIds\":[\"Out1\",\"Out2\"],\"side\":\"RIGHT\"},\"type\":\"ConnectorPlacement.EquallySpacedRectSide\",\"uuid\":\"c3dbff62-2cbb-49e5-a718-27c684f0604c\"},{\"content\":{\"connectorIds\":[\"In1\"],\"side\":\"TOP\"},\"type\":\"ConnectorPlacement.EquallySpacedRectSide\",\"uuid\":\"83a064d4-85ee-4dcc-804e-22587799da9e\"}]},\"type\":\"ConnectorPlacement.EquallySpacedConnector\",\"uuid\":\"6d33be0e-4d36-4c84-a292-f5ef4e252a8e\"}],\"packageUris\":[\"http://schema.mathworks.com/mf0/Connector/R2020b\"],\"version\":\"1.0\"}"
  Vectoring7 : Subsystem  Commented=on
      settings: PortSchema="{\"entries\":[{\"content\":{\"sides\":[{\"content\":{\"connectorIds\":[]},\"type\":\"ConnectorPlacement.EquallySpacedRectSide\",\"uuid\":\"7f0919a1-928c-4229-a557-ae6b37c0e18a\"},{\"content\":{\"connectorIds\":[\"Out1\",\"Out2\"],\"side\":\"RIGHT\"},\"type\":\"ConnectorPlacement.EquallySpacedRectSide\",\"uuid\":\"c3dbff62-2cbb-49e5-a718-27c684f0604c\"},{\"content\":{\"connectorIds\":[\"In1\"],\"side\":\"TOP\"},\"type\":\"ConnectorPlacement.EquallySpacedRectSide\",\"uuid\":\"83a064d4-85ee-4dcc-804e-22587799da9e\"}]},\"type\":\"ConnectorPlacement.EquallySpacedConnector\",\"uuid\":\"6d33be0e-4d36-4c84-a292-f5ef4e252a8e\"}],\"packageUris\":[\"http://schema.mathworks.com/mf0/Connector/R2020b\"],\"version\":\"1.0\"}"
  Vectoring8 : Subsystem  Commented=on
      settings: PortSchema="{\"entries\":[{\"content\":{\"sides\":[{\"content\":{\"connectorIds\":[]},\"type\":\"ConnectorPlacement.EquallySpacedRectSide\",\"uuid\":\"7f0919a1-928c-4229-a557-ae6b37c0e18a\"},{\"content\":{\"connectorIds\":[\"Out1\",\"Out2\"],\"side\":\"RIGHT\"},\"type\":\"ConnectorPlacement.EquallySpacedRectSide\",\"uuid\":\"c3dbff62-2cbb-49e5-a718-27c684f0604c\"},{\"content\":{\"connectorIds\":[\"In1\",\"In2\"],\"side\":\"TOP\"},\"type\":\"ConnectorPlacement.EquallySpacedRectSide\",\"uuid\":\"83a064d4-85ee-4dcc-804e-22587799da9e\"},{\"content\":{\"connectorIds\":[\"Out3\"],\"side\":\"BOTTOM\"},\"type\":\"ConnectorPlacement.EquallySpacedRectSide\",\"uuid\":\"eea76909-33f2-4847-bfa0-f6ca22c12ff2\"}]},\"type\":\"ConnectorPlacement.EquallySpacedConnector\",\"uuid\":\"6d33be0e-4d36-4c84-a292-f5ef4e252a8e\"}],\"packageUris\":[\"http://schema.mathworks.com/mf0/Connector/R2020b\"],\"version\":\"1.0\"}"
  Vectoring9 : Subsystem  Commented=on
      settings: PortSchema="{\"entries\":[{\"content\":{\"sides\":[{\"content\":{\"connectorIds\":[]},\"type\":\"ConnectorPlacement.EquallySpacedRectSide\",\"uuid\":\"7f0919a1-928c-4229-a557-ae6b37c0e18a\"},{\"content\":{\"connectorIds\":[\"Out1\",\"Out2\"],\"side\":\"RIGHT\"},\"type\":\"ConnectorPlacement.EquallySpacedRectSide\",\"uuid\":\"c3dbff62-2cbb-49e5-a718-27c684f0604c\"},{\"content\":{\"connectorIds\":[\"In1\",\"In2\"],\"side\":\"TOP\"},\"type\":\"ConnectorPlacement.EquallySpacedRectSide\",\"uuid\":\"83a064d4-85ee-4dcc-804e-22587799da9e\"},{\"content\":{\"connectorIds\":[\"Out3\"],\"side\":\"BOTTOM\"},\"type\":\"ConnectorPlacement.EquallySpacedRectSide\",\"uuid\":\"eea76909-33f2-4847-bfa0-f6ca22c12ff2\"}]},\"type\":\"ConnectorPlacement.EquallySpacedConnector\",\"uuid\":\"6d33be0e-4d36-4c84-a292-f5ef4e252a8e\"}],\"packageUris\":[\"http://schema.mathworks.com/mf0/Connector/R2020b\"],\"version\":\"1.0\"}"
  Vitis HLS : hdlBasic/Vitis HLS  Commented=on  anytable='C:\ELEC522\jz118\HLS\cordic\solution1'  fast_sim=off  display_datatype=off  rate_propagation_method=Simulink system period  model_file_path=''  latency=1  block_type=vitis_hls
      settings: infoedit=This block allows including C,C++ and SystemC source files in System Generator for DSP designs.
  Vitis HLS1 : hdlBasic/Vitis HLS  Commented=on  anytable='C:\ELEC522\jz118\HLS\cordic\solution1'  fast_sim=off  display_datatype=off  rate_propagation_method=Simulink system period  model_file_path=''  latency=1  block_type=vitis_hls
      settings: infoedit=This block allows including C,C++ and SystemC source files in System Generator for DSP designs.
  Vitis HLS2 : hdlBasic/Vitis HLS  Commented=on  anytable='C:\ELEC522\jz118\HLS\cordic\solution1'  fast_sim=off  display_datatype=off  rate_propagation_method=Simulink system period  model_file_path=''  latency=1  block_type=vitis_hls
      settings: infoedit=This block allows including C,C++ and SystemC source files in System Generator for DSP designs.
  ctrl : hdlBasic/Gateway In  gui_display_data_type=Boolean  arith_type=Boolean  n_bits=16  bin_pt=13  preci_type=Single  exp_width=8  frac_width=24  rows=1  columns=1  quantization="Round  (unbiased: +/- Inf)"  overflow=Saturate  period=1  UseAsADC=off  ADCChannel='1'  interface=AXI4-Lite  automatic_assignment=on  address_offset=hex2dec('00')  intf_name=''  intf_description='ctrl_t'  default_value=0  timing_constraint=None  locs_specified=off  LOCs={}  io_standard={}  inherit_from_input=off  hdl_port=on  XmcBlockStatus=1  maskContainerNames=group4  block_type=gatewayin  block_config=sysgen:gateway_in_config  block_width_w=590  block_height_w=620  block_width=640  block_height=850
  ctrl1 : hdlBasic/Gateway In  Commented=on  gui_display_data_type=Boolean  arith_type=Boolean  n_bits=16  bin_pt=13  preci_type=Single  exp_width=8  frac_width=24  rows=1  columns=1  quantization="Round  (unbiased: +/- Inf)"  overflow=Saturate  period=1  UseAsADC=off  ADCChannel='1'  interface=AXI4-Lite  automatic_assignment=on  address_offset=hex2dec('00')  intf_name=''  intf_description='ctrl_t'  default_value=0  timing_constraint=None  locs_specified=off  LOCs={}  io_standard={}  inherit_from_input=off  hdl_port=on  XmcBlockStatus=1  maskContainerNames=group4  block_type=gatewayin  block_config=sysgen:gateway_in_config  block_width_w=590  block_height_w=620  block_width=640  block_height=850
  wires:
  Gateway In1/1 -> Vitis HLS/2
  Constant2/1 -> Gateway In1/1
  Gateway In9/1 -> Vitis HLS/6
  Gateway In3/1 -> Vitis HLS/3
  Gateway In4/1 -> Scope3/1, Vitis HLS/5
  Gateway In2/1 -> Vitis HLS/4
  Vitis HLS/1 -> Gateway Out/1
  Vitis HLS/2 -> Gateway Out1/1
  Vitis HLS/3 -> Gateway Out2/1
  Vitis HLS/4 -> Gateway Out3/1
  Vitis HLS/5 -> Gateway Out4/1
  Vitis HLS/6 -> Gateway Out5/1
  Vitis HLS/7 -> Gateway Out6/1
  Gateway Out6/1 -> Scope/1
  Gateway Out7/1 -> Scope/2
  Vitis HLS/8 -> Mux/1, Gateway Out7/1
  Vitis HLS/9 -> Gateway Out8/1
  Gateway Out8/1 -> Scope1/1
  Vitis HLS/10 -> Gateway Out9/1
  Vitis HLS/11 -> Gateway Out10/1
  Gateway Out10/1 -> Scope6/1
  From Workspace4/1 -> Gateway In3/1
  From Workspace1/1 -> Gateway In2/1
  From Workspace2/1 -> Gateway In9/1
  From Workspace3/1 -> Gateway In4/1
  Vectoring/1(Out1) -> Rotation/1(In3)
  From Workspace8/1 -> Rotation2/2(In2)
  From Workspace7/1 -> Rotation1/2(In2)
  From Workspace6/1 -> Rotation/2(In2)
  From Workspace5/1 -> Vectoring/1(In2)
  Gateway Out11/1 -> To Workspace/1
  Gateway Out12/1 -> To Workspace1/1
  Gateway Out14/1 -> To Workspace2/1
  Gateway Out13/1 -> To Workspace3/1
  Rotation1/1(Out1) -> Rotation2/1(In3)
  Rotation2/1(Out1) -> Gateway Out11/1
  Rotation/1(Out1) -> Rotation1/1(In3)
  Rotation/2(Out9) -> Vectoring1/1(In2)
  Rotation1/2(Out9) -> Rotation3/2(In2)
  Rotation2/2(Out9) -> Rotation4/2(In2)
  Vectoring1/1(Out1) -> Rotation3/1(In3)
  Rotation4/1(Out1) -> Gateway Out12/1
  Rotation3/1(Out1) -> Rotation4/1(In3)
  Rotation3/2(Out9) -> Gateway Out13/1
  Rotation4/2(Out9) -> Gateway Out14/1
  From Workspace9/1 -> Vectoring2/1(In2)
  From Workspace10/1 -> Rotation5/2(In2)
  Vitis HLS/12 -> Gateway Out16/1
  Gateway Out16/1 -> Scope6/2
  Gateway Out9/1 -> Scope1/2
  Gateway Out5/1 -> Terminator/1
  Gateway Out4/1 -> Terminator1/1
  Gateway Out3/1 -> Terminator2/1
  Gateway Out2/1 -> Terminator3/1
  Gateway Out1/1 -> Terminator4/1
  Mux/1 -> Vitis HLS/1
  Constant/1 -> Mux/2
  Constant1/1 -> Mux/3
  Gateway Out/1 -> Scope/3
  Gateway Out17/1 -> Scope2/3
  Vitis HLS1/10 -> Gateway Out28/1
  Gateway Out22/1 -> Terminator7/1
  Gateway Out21/1 -> Terminator8/1
  Gateway Out24/1 -> Terminator5/1
  Gateway Out18/1 -> Terminator9/1
  Gateway Out28/1 -> Scope7/2
  From Workspace14/1 -> Gateway In7/1
  Gateway Out20/1 -> Scope9/2
  Vitis HLS1/7 -> Gateway Out25/1
  Gateway Out19/1 -> Scope9/1
  Gateway In8/1 -> Scope8/1, Vitis HLS1/5
  Gateway In6/1 -> Vitis HLS1/4
  From Workspace13/1 -> Gateway In8/1
  Vitis HLS1/8 -> Gateway Out26/1
  From Workspace12/1 -> Gateway In10/1
  Gateway In5/1 -> Vitis HLS1/2
  Gateway Out27/1 -> Scope7/1
  Vitis HLS1/11 -> Gateway Out19/1
  Gateway Out26/1 -> Scope2/2
  From Workspace11/1 -> Gateway In6/1
  Gateway Out25/1 -> Scope2/1
  Vitis HLS1/4 -> Gateway Out22/1
  Vitis HLS1/12 -> Gateway Out20/1
  Vitis HLS1/6 -> Gateway Out24/1
  Vitis HLS1/3 -> Gateway Out21/1
  Vitis HLS1/2 -> Gateway Out18/1
  Gateway In7/1 -> Vitis HLS1/3
  Gateway In10/1 -> Vitis HLS1/6
  Vitis HLS1/5 -> Gateway Out23/1
  Constant5/1 -> Gateway In5/1
  Vitis HLS1/9 -> Gateway Out27/1
  Vitis HLS1/1 -> Gateway Out17/1
  Gateway Out23/1 -> Terminator6/1
  Constant3/1 -> Gateway In11/1
  Gateway In11/1 -> Vitis HLS1/1
  Vectoring2/1(Out1) -> Rotation5/1(In3)
  Vectoring3/1(Out1) -> Rotation6/1(In3)
  Rotation5/2(Out9) -> Vectoring3/1(In2)
  Rotation5/1(Out1) -> Rotation7/1(In3)
  Rotation6/1(Out1) -> Rotation9/1(In3)
  Rotation8/2(Out9) -> Rotation9/2(In2)
  Rotation7/1(Out1) -> Rotation8/1(In3)
  From Workspace15/1 -> Rotation7/2(In2)
  From Workspace16/1 -> Rotation8/2(In2)
  Rotation7/2(Out9) -> Rotation6/2(In2)
  Gateway Out29/1 -> To Workspace5/1
  Rotation9/1(Out1) -> Gateway Out29/1
  Gateway Out15/1 -> To Workspace4/1
  Rotation8/1(Out1) -> Gateway Out15/1
  Gateway Out31/1 -> To Workspace6/1
  Gateway Out30/1 -> To Workspace7/1
  Rotation6/2(Out9) -> Gateway Out30/1
  Rotation9/2(Out9) -> Gateway Out31/1
  Vectoring4/1(Out1) -> Scope24/1, Rotation10/1(In3), Scope11/2
  From Workspace18/1 -> Gateway In12/1
  Gateway In12/1 -> Scope11/1, Rotation10/2(In2)
  Rotation12/1(Out1) -> Scope15/1, Gateway Out32/1
  Gateway Out32/1 -> To Workspace8/1
  Rotation10/1(Out1) -> Rotation11/1(In3), Scope4/2
  Rotation11/1(Out1) -> Rotation12/1(In3), Scope5/2
  Gateway In13/1 -> Scope4/1, Rotation11/2(In2)
  From Workspace19/1 -> Gateway In13/1
  From Workspace20/1 -> Gateway In14/1
  Gateway In14/1 -> Scope5/1, Rotation12/2(In2)
  Rotation14/1(Out1) -> Rotation15/1(In3)
  Rotation12/2(Out9) -> Rotation15/2(In2)
  Rotation11/2(Out9) -> Rotation14/2(In2)
  Rotation10/2(Out9) -> Vectoring5/1(In2)
  From Workspace17/1 -> Gateway In15/1
  Gateway In15/1 -> Scope10/1, Vectoring4/1(In2)
  Vectoring5/1(Out1) -> Rotation14/1(In3)
  Rotation15/1(Out1) -> Scope12/1, Gateway Out33/1
  Gateway Out33/1 -> To Workspace9/1
  Gateway Out34/1 -> To Workspace10/1
  Rotation15/2(Out9) -> Scope13/1, Gateway Out34/1
  Gateway Out35/1 -> To Workspace11/1
  Rotation10/3(Out2) -> Scope11/3
  Rotation14/2(Out9) -> Scope14/1, Gateway Out35/1
  From Workspace21/1 -> Gateway In16/1
  From Workspace22/1 -> Scope17/1, Gateway In17/1
  Register/1 -> Gateway Out36/1
  Gateway Out36/1 -> Scope16/1
  Gateway In16/1 -> Register/2
  Gateway In17/1 -> Register/1
  From Workspace23/1 -> Gateway In18/1
  Gateway In18/1 -> Vectoring6/1(In2)
  Gateway Out37/1 -> Scope18/1
  From Workspace24/1 -> Gateway In19/1
  Gateway In19/1 -> Rotation13/2(In2)
  Rotation13/1(Out1) -> Gateway Out37/1
  Rotation13/3(Out2) -> Scope19/1
  Rotation13/2(Out9) -> Vectoring7/1(In2)
  Gateway Out38/1 -> Scope20/1
  Vectoring6/1(Out1) -> Rotation13/1(In3)
  Vectoring7/1(Out1) -> Gateway Out38/1
  Vectoring6/2(Out2) -> Scope21/1
  Rotation13/4(Out3) -> Negate/1
  Vectoring7/2(Out2) -> Scope23/1
  Negate/1 -> Scope22/1
  Rotation16/5(Out3) -> Scope29/1
  Rotation16/4(Out9) -> Vectoring9/2(In2)
  From Workspace26/1 -> Gateway In21/1
  From Workspace25/1 -> Gateway In20/1
  Gateway In21/1 -> Rotation16/3(In2)
  Gateway In20/1 -> Vectoring8/2(In2)
  Vectoring8/1(Out1) -> Rotation16/1(In3)
  Rotation19/3(Out2) -> Terminator11/1
  Rotation18/3(Out2) -> Terminator12/1
  Rotation20/3(Out2) -> Terminator13/1
  Rotation21/3(Out2) -> Terminator14/1
  Rotation17/3(Out9) -> Rotation18/2(In2)
  Rotation18/1(Out1) -> Rotation20/1(In3)
  Rotation19/2(Out9) -> Rotation20/2(In2)
  Rotation18/2(Out9) -> Vectoring10/1(In2)
  Rotation20/2(Out9) -> Rotation21/2(In2)
  Rotation21/2(Out9) -> Scope46/1, Vectoring11/1(In2)
  Vectoring10/1(Out1) -> Rotation21/1(In3)
  Vectoring11/1(Out1) -> Gateway Out42/1
  Gateway Out42/1 -> Scope32/1
  Vectoring10/2(Out2) -> Scope33/1
  Rotation21/4(Out3) -> Scope34/1
  Vectoring11/2(Out2) -> Scope35/1
  Rotation20/4(Out3) -> Scope36/1
  Rotation18/4(Out3) -> Scope37/1
  Rotation19/4(Out3) -> Scope38/1
  From Workspace27/1 -> Gateway In22/1
  From Workspace28/1 -> Gateway In23/1
  Gateway In23/1 -> Rotation19/2(In2)
  Gateway Out41/1 -> To Workspace17/1
  Rotation33/1(Out1) -> Gateway Out41/1
  Rotation32/1(Out1) -> Gateway Out40/1
  Rotation31/1(Out1) -> Gateway Out39/1
  Gateway Out40/1 -> To Workspace18/1
  Gateway Out39/1 -> To Workspace19/1
  Rotation19/1(Out1) -> Rotation22/1(In3)
  Rotation22/1(Out1) -> Rotation25/1(In3)
  Rotation25/1(Out1) -> Rotation28/1(In3)
  Rotation28/1(Out1) -> Rotation31/1(In3)
  Rotation22/2(Out9) -> Rotation23/2(In2)
  Rotation25/2(Out9) -> Rotation26/2(In2)
  Rotation28/2(Out9) -> Rotation29/2(In2)
  Rotation31/2(Out9) -> Rotation32/2(In2)
  Rotation20/1(Out1) -> Rotation23/1(In3)
  Rotation23/1(Out1) -> Rotation26/1(In3)
  Rotation26/1(Out1) -> Rotation29/1(In3)
  Rotation29/1(Out1) -> Rotation32/1(In3)
  Rotation24/1(Out1) -> Rotation27/1(In3)
  Rotation27/1(Out1) -> Rotation30/1(In3)
  Rotation30/1(Out1) -> Rotation33/1(In3)
  Rotation21/1(Out1) -> Rotation24/1(In3)
  Rotation23/2(Out9) -> Rotation24/2(In2)
  Rotation26/2(Out9) -> Rotation27/2(In2)
  Rotation29/2(Out9) -> Rotation30/2(In2)
  Rotation32/2(Out9) -> Rotation33/2(In2)
  Rotation22/3(Out2) -> Terminator15/1
  Rotation25/3(Out2) -> Terminator16/1
  Rotation28/3(Out2) -> Terminator17/1
  Rotation31/3(Out2) -> Terminator18/1
  Rotation32/3(Out2) -> Terminator19/1
  Rotation29/3(Out2) -> Terminator20/1
  Rotation26/3(Out2) -> Terminator21/1
  Rotation23/3(Out2) -> Terminator22/1
  Rotation33/3(Out2) -> Terminator23/1
  Rotation30/3(Out2) -> Terminator24/1
  Rotation27/3(Out2) -> Terminator25/1
  Rotation24/3(Out2) -> Terminator26/1
  From Workspace29/1 -> Gateway In24/1
  Gateway In24/1 -> Rotation22/2(In2)
  Gateway In25/1 -> Rotation25/2(In2)
  From Workspace30/1 -> Gateway In25/1
  Gateway In26/1 -> Rotation28/2(In2)
  From Workspace31/1 -> Gateway In26/1
  Gateway In27/1 -> Rotation31/2(In2)
  From Workspace32/1 -> Gateway In27/1
  Gateway Out44/1 -> To Workspace16/1
  Rotation33/2(Out9) -> Gateway Out44/1
  Gateway Out45/1 -> To Workspace15/1
  Rotation30/2(Out9) -> Gateway Out45/1
  Gateway Out46/1 -> To Workspace14/1
  Rotation27/2(Out9) -> Gateway Out46/1
  Gateway Out47/1 -> Scope25/1, To Workspace13/1
  Rotation24/2(Out9) -> Gateway Out47/1
  Rotation24/4(Out3) -> Scope27/1
  Rotation23/4(Out3) -> Scope31/1
  Rotation22/4(Out3) -> Scope40/1
  Rotation25/4(Out3) -> Scope41/1
  Rotation28/4(Out3) -> Scope42/1
  Rotation31/4(Out3) -> Scope43/1
  Rotation26/4(Out3) -> Scope44/1
  Rotation29/4(Out3) -> Scope45/1
  Rotation32/4(Out3) -> Scope47/1
  Rotation27/4(Out3) -> Scope48/1
  Rotation30/4(Out3) -> Scope49/1
  Rotation33/4(Out3) -> Scope50/1
  Vectoring8/3(Out2) -> Scope28/1
  From Workspace33/1 -> Gateway In28/1
  Gateway In28/1 -> Vectoring8/1(In1)
  Vectoring8/2(Out3) -> Rotation16/2(In1)
  Rotation16/2(Out4) -> Rotation17/2(In1)
  Rotation16/1(Out1) -> Rotation17/1(In3)
  Gateway In22/1 -> Rotation17/3(In2)
  Rotation17/4(Out3) -> Scope26/1
  Rotation16/3(Out2) -> Vectoring9/1(In1)
  Vectoring9/3(Out2) -> Scope30/1
  From Workspace38/1 -> ctrl/1
  ctrl/1 -> Vectoring14/1(In1)
  Rotation34/3(Out2) -> Vectoring15/1(In1)
  Rotation34/4(Out9) -> Vectoring15/2(In2)
  Gateway In32/1 -> Rotation36/3(In2)
  Vectoring14/2(Out3) -> Rotation34/2(In1)
  From Workspace36/1 -> Gateway In31/1
  From Workspace37/1 -> Gateway In32/1
  From Workspace34/1 -> Gateway In29/1
  Gateway In29/1 -> Vectoring14/2(In2)
  Gateway In30/1 -> Rotation34/3(In2)
  Vectoring14/1(Out1) -> Rotation34/1(In3)
  From Workspace35/1 -> Gateway In30/1
  Gateway In31/1 -> Rotation35/3(In2)
  Rotation34/1(Out1) -> Rotation35/1(In3)
  Rotation34/2(Out4) -> Rotation35/2(In1)
  Rotation35/1(Out1) -> Rotation36/1(In3)
  Rotation35/2(Out4) -> Rotation36/2(In1)
  Rotation36/5(Out3) -> Scope54/1
  Vectoring15/1(Out1) -> Rotation37/1(In3)
  Vectoring15/2(Out3) -> Rotation37/2(In1)
  Rotation37/3(Out2) -> Vectoring12/1(In1)
  Rotation37/4(Out9) -> Vectoring12/2(In2)
  Vectoring12/3(Out2) -> Scope55/1
  Rotation37/5(Out3) -> Scope56/1
  Rotation37/1(Out1) -> Rotation38/1(In3)
  Rotation37/2(Out4) -> Rotation38/2(In1)
  Rotation38/5(Out3) -> Scope57/1
  Vectoring12/1(Out1) -> Rotation39/1(In3)
  Vectoring12/2(Out3) -> Rotation39/2(In1)
  Rotation39/5(Out3) -> Scope58/1
  Rotation35/4(Out9) -> Rotation37/3(In2)
  Rotation36/4(Out9) -> Rotation38/3(In2)
  Rotation38/4(Out9) -> Rotation39/3(In2)
  Rotation36/3(Out2) -> Terminator10/1
  Rotation35/3(Out2) -> Terminator27/1
  Rotation38/3(Out2) -> Terminator28/1
  Rotation39/1(Out1) -> Rotation48/1(In3)
  Rotation39/2(Out4) -> Rotation48/2(In1)
  Rotation39/4(Out9) -> Mux1/3
  Constant11/1 -> Mux1/2
  Mux1/1 -> Negate1/1
  Rotation39/3(Out2) -> Mux1/1
  Rotation36/1(Out1) -> Rotation40/1(In3)
  Rotation36/2(Out4) -> Rotation40/2(In1)
  Rotation40/5(Out3) -> Scope59/1
  Gateway In37/1 -> Rotation43/3(In2)
  Gateway In36/1 -> Rotation42/3(In2)
  From Workspace41/1 -> Gateway In36/1
  From Workspace39/1 -> Gateway In34/1
  Gateway In34/1 -> Rotation40/3(In2)
  Gateway In35/1 -> Rotation41/3(In2)
  From Workspace40/1 -> Gateway In35/1
  From Workspace42/1 -> Gateway In37/1
  Rotation40/1(Out1) -> Rotation41/1(In3)
  Rotation40/2(Out4) -> Rotation41/2(In1)
  Rotation41/1(Out1) -> Rotation42/1(In3)
  Rotation41/2(Out4) -> Rotation42/2(In1)
  Rotation42/1(Out1) -> Rotation43/1(In3)
  Rotation42/2(Out4) -> Rotation43/2(In1)
  Rotation41/5(Out3) -> Scope60/1
  Rotation42/5(Out3) -> Scope61/1
  Rotation43/5(Out3) -> Scope62/1
  Rotation38/1(Out1) -> Rotation44/1(In3)
  Rotation38/2(Out4) -> Rotation44/2(In1)
  Rotation44/1(Out1) -> Rotation45/1(In3)
  Rotation44/2(Out4) -> Rotation45/2(In1)
  Rotation45/1(Out1) -> Rotation46/1(In3)
  Rotation45/2(Out4) -> Rotation46/2(In1)
  Rotation46/1(Out1) -> Rotation47/1(In3)
  Rotation46/2(Out4) -> Rotation47/2(In1)
  Rotation40/4(Out9) -> Rotation44/3(In2)
  Rotation41/4(Out9) -> Rotation45/3(In2)
  Rotation42/4(Out9) -> Rotation46/3(In2)
  Rotation43/4(Out9) -> Rotation47/3(In2)
  Rotation40/3(Out2) -> Terminator29/1
  Rotation41/3(Out2) -> Terminator30/1
  Rotation42/3(Out2) -> Terminator31/1
  Rotation43/3(Out2) -> Terminator32/1
  Rotation44/3(Out2) -> Terminator33/1
  Rotation45/3(Out2) -> Terminator34/1
  Rotation46/3(Out2) -> Terminator35/1
  Rotation47/3(Out2) -> Terminator36/1
  Rotation44/5(Out3) -> Scope63/1
  Rotation45/5(Out3) -> Scope64/1
  Rotation46/5(Out3) -> Scope66/1
  Rotation47/5(Out3) -> Scope67/1
  Rotation47/4(Out9) -> Rotation51/3(In2)
  Rotation46/4(Out9) -> Rotation50/3(In2)
  Rotation45/4(Out9) -> Rotation49/3(In2)
  Rotation44/4(Out9) -> Rotation48/3(In2)
  Rotation48/1(Out1) -> Rotation49/1(In3)
  Rotation48/2(Out4) -> Rotation49/2(In1)
  Rotation49/2(Out4) -> Rotation50/2(In1)
  Rotation49/1(Out1) -> Rotation50/1(In3)
  Rotation50/2(Out4) -> Rotation51/2(In1)
  Rotation50/1(Out1) -> Rotation51/1(In3)
  Rotation48/5(Out3) -> Scope68/1
  Rotation49/5(Out3) -> Scope69/1
  Rotation50/5(Out3) -> Scope70/1
  Rotation51/5(Out3) -> Scope71/1
  Rotation43/1(Out1) -> Terminator37/1
  Rotation43/2(Out4) -> Terminator38/1
  Rotation47/1(Out1) -> Terminator39/1
  Rotation47/2(Out4) -> Terminator40/1
  Rotation51/1(Out1) -> Terminator41/1
  Rotation51/2(Out4) -> Terminator42/1
  Gateway Out43/1 -> Scope65/1, To Workspace12/1
  Gateway Out48/1 -> Scope72/1, To Workspace20/1
  Constant4/1 -> Mux2/2
  Rotation48/4(Out9) -> Mux2/3
  Rotation48/3(Out2) -> Mux2/1
  Gateway Out49/1 -> Scope73/1, To Workspace21/1
  Constant6/1 -> Mux3/2
  Rotation49/4(Out9) -> Mux3/3
  Rotation49/3(Out2) -> Mux3/1
  Gateway Out50/1 -> Scope74/1, To Workspace22/1
  Constant7/1 -> Mux4/2
  Rotation50/4(Out9) -> Mux4/3
  Rotation50/3(Out2) -> Mux4/1
  Gateway Out51/1 -> Scope75/1, To Workspace23/1
  Constant8/1 -> Mux5/2
  Rotation51/4(Out9) -> Mux5/3
  Rotation51/3(Out2) -> Mux5/1
  Negate1/1 -> Gateway Out43/1
  Mux2/1 -> Negate2/1
  Negate2/1 -> Gateway Out48/1
  Mux3/1 -> Negate3/1
  Negate3/1 -> Gateway Out49/1
  Mux4/1 -> Negate4/1
  Negate4/1 -> Gateway Out50/1
  Mux5/1 -> Negate5/1
  Negate5/1 -> Gateway Out51/1
  Vectoring15/3(Out2) -> Terminator45/1
  From Workspace43/1 -> Gateway In33/1
  From Workspace44/1 -> ctrl1/1
  Gateway Out52/1 -> To Workspace24/1
  Gateway In33/1 -> Vitis HLS2/4
  Vitis HLS2/4 -> Terminator47/1
  Vitis HLS2/5 -> Terminator52/1
  Vitis HLS2/6 -> Terminator51/1
  Vitis HLS2/2 -> Terminator43/1
  Vitis HLS2/9 -> Terminator49/1
  Constant12/1 -> Vitis HLS2/1, Vitis HLS2/6
  Vitis HLS2/1 -> Terminator48/1
  Constant9/1 -> Mux6/2
  Constant10/1 -> Vitis HLS2/5
  Mux6/1 -> Gateway Out52/1
  Constant13/1 -> Vitis HLS2/2
  Vitis HLS2/3 -> Terminator46/1
  Vitis HLS2/8 -> Terminator53/1
  Constant14/1 -> Vitis HLS2/3
  Vitis HLS2/7 -> Terminator54/1
  Vitis HLS2/10 -> Mux6/3
  Vitis HLS2/11 -> Mux6/1
